simulink model "fft32kpt_ssr32_float"  (R2024a)
settings: Solver=VariableStepAuto  StartTime=0.0  StopTime=sample_period*N*6  RelTol=1e-3
PreLoadFcn:
  | clk_freq = 570e6;
  | SSR=32; % transpose block SSR settings...
  | sample_period = 1/(SSR*clk_freq);
  | N=32768; % fft point size
  | binw=(1/sample_period) / (2*N); % bin width
  | bin_freq = 2*pi*3*binw+pi*binw; % sin, cos freq centered in channel
  | 
  | % for transpose block
  | DATA_WIDTH=32;
  | M=32;
  | N1=N/M;
  | MEM_STYLE=4; % MEM OPTIONS: 4 - ULTRA, 0 - AUTO, 1 - BRAM, 5 - MIXED
InitFcn:
  | clk_freq = 570e6;
  | SSR=32; % transpose block SSR settings...
  | sample_period = 1/(SSR*clk_freq);
  | N=32768; % fft point size
  | binw=(1/sample_period) / (2*N); % bin width
  | bin_freq = 2*pi*3*binw+pi*binw; % sin, cos freq centered in channel
  | 
  | % for transpose block
  | DATA_WIDTH=32;
  | M=32;
  | N1=N/M;
  | MEM_STYLE=4; % MEM OPTIONS: 4 - ULTRA, 0 - AUTO, 1 - BRAM, 5 - MIXED
undefined symbols (not defined in the file or in its folder): None, S, vsva2197, xcvc1902
libraries: hdlBasic x139, aieBasic x95, aieUtilities x32, aieDSP x32, hdlUtilities x32, matrix_library x32, hdlSSR x12, hdlDSPIP x1, simulink x1, dspxfrm3 x1, vmcUtilities x1
(part 2 of 4)

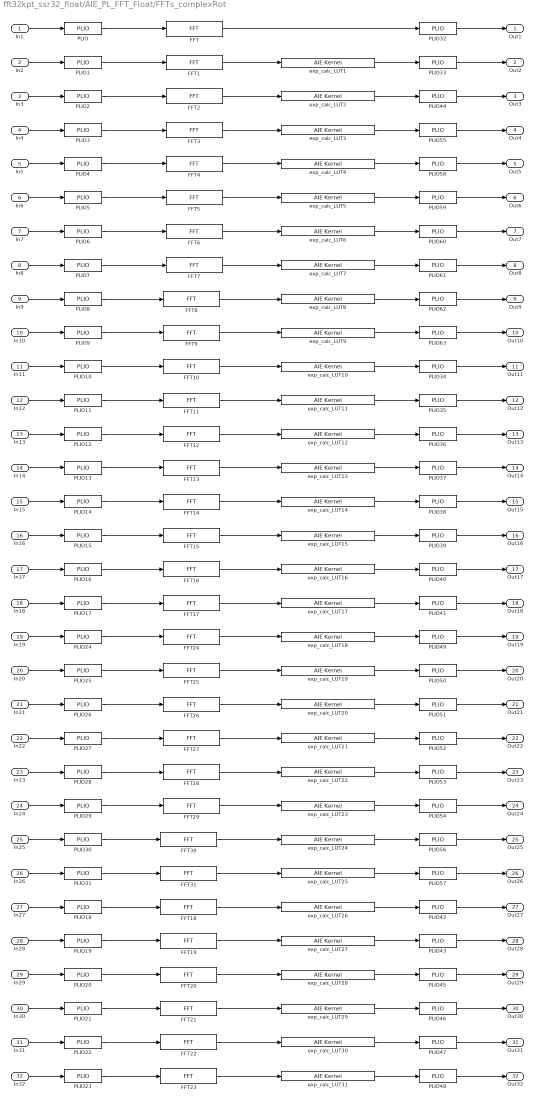
== system fft32kpt_ssr32_float/AIE_PL_FFT_Float/FFTs_complexRot ==
  In1 : Inport
  In2 : Inport  Port=2
  In3 : Inport  Port=3
  In4 : Inport  Port=4
  In5 : Inport  Port=5
  In6 : Inport  Port=6
  In7 : Inport  Port=7
  In8 : Inport  Port=8
  In9 : Inport  Port=9
  In10 : Inport  Port=10
  In11 : Inport  Port=11
  In12 : Inport  Port=12
  In13 : Inport  Port=13
  In14 : Inport  Port=14
  In15 : Inport  Port=15
  In16 : Inport  Port=16
  In17 : Inport  Port=17
  In18 : Inport  Port=18
  In19 : Inport  Port=19
  In20 : Inport  Port=20
  In21 : Inport  Port=21
  In22 : Inport  Port=22
  In23 : Inport  Port=23
  In24 : Inport  Port=24
  In25 : Inport  Port=25
  In26 : Inport  Port=26
  In27 : Inport  Port=27
  In28 : Inport  Port=28
  In29 : Inport  Port=29
  In30 : Inport  Port=30
  In31 : Inport  Port=31
  In32 : Inport  Port=32
  FFT{,1..31} (32 alike) : aieDSP/FFT  AIE_VARIANT=1  data_type=cfloat  data_out_type=cfloat  twiddle_type=cfloat  point_size=N/32  input_window_size=N/32  shift_val=0  rnd_mode=Round symmetrical to infinity  sat_mode=0-None  ssr=1  twiddle_mode=0  use_ssr_widget_kernels=off  casc_length=3  transform_fft_nifft=1  TP_API=0  TP_DYN_PT_SIZE=0  blockJsonConstraints=[]  blockJsonConstraintsInternal=[]  spec=vmc_fft.json  SerializedMaskParamNames=[]  SerializedMaskParamValues=[]  SerializedMaskParamVisibilities=[]  block_type=FFT  SerializedMaskParamDataypes=uint|typename|typename|typename|uint|uint|uint|uint|uint|uint|uint|uint|uint|uint|uint|uint  SerializedMaskParamEnumStrArr=0|0|0|0|0|0|0|Round to positive infinity,Round to negative infinity,Round symmetrical to infinity,Round symmetrical to zero,Round convergent to even,Round convergent to odd|0-None,1-Asymmetric,3-Symmetric|0|0|0|0|0|0|0  SerializedMaskParamEnumValArr=0|0|0|0|0|0|0|2,3,4,5,6,7|0,1,3|0|0|0|0|0|0|0  SerializedMaskParamVectorArr=0|0|0|0|0|0|0|0|0|0|0|0|0|0|0|0  SerializedMaskParamKeys=AIE_VARIANT|TT_DATA|TT_OUT_DATA|TT_TWIDDLE|TP_POINT_SIZE|TP_WINDOW_VSIZE|TP_SHIFT|TP_RND|TP_SAT|TP_PARALLEL_POWER|TP_TWIDDLE_MODE|TP_USE_WIDGETS|TP_CASC_LEN|TP_FFT_NIFFT|TP_API|TP_DYN_PT_SIZE
  PLIO{,1..63} (64 alike) : aieBasic/PLIO  PlioWidth=64  PlioFreqSpec=on  PlioFreq=clk_freq/1e6  ColLocation=0  channel=0  blockJsonConstraints=[]  deprecateConstraints=0
  exp_calc_LUT1 : aieBasic/AIE Kernel  KernelAllAttrs=|  PortNames={'cb_input1'; 'cb_output1'}  PortSerializedTypes={'{Q2{R{Tadf::input_buffer{1{t{Scfloat}}}}}}'; '{Q2{P{Toutput_stream{1{t{Scfloat}}}}}}'}  PortWindowSizes={1.024000000000000000e+03, 0.000000000000000000e+00}  PortWindowMargins={0.000000000000000000e+00, 0.000000000000000000e+00}  PortSynchronicities={'sync', 'auto'}  PortSignalSizes={0.000000000000000000e+00; 1.024000000000000000e+03}  FunctionTemplateSpecKind=implicit  FunctionTemplateParamNames={'PHASE_INDEX'}  FunctionTemplateParamKinds={'nontype'}  FunctionTemplateParamTypes={'unsigned int'}  FunctionTemplateParamValues={'1'}  FunctionIndex=1  FunctionTabVisible=on  FunctionTemplateParamsVisible=on  FunctionDeclTypeOptions=|  FunctionDecl=|  FunctionTemplateParams={ 'PHASE_INDEX', 'unsigned int', '1' }  FunctionTemplateParamsEnables={'off', 'off', 'on'}  PortAttrs={ 'input', 'cb_input1', 'adf::input_buffer< cfloat > & restrict', '1024', '0', 'sync', ''; 'output', 'cb_output1', 'output_stream_cfloat * restrict', '', '', '', '1024' }  PortAttrsEnables={'off', 'off', 'off', 'on', 'off', 'off', 'off';'off', 'off', 'off', 'off', 'off', 'off', 'on'}  SampleTime=-1  KernelHeaderFile=exp_calc_float.h  KernelFunction=exp_calc_float_lookup  KernelSourceFile=exp_calc_float.cc  KernelSearchPaths={}  PreProcOptions={}  blockJsonConstraints=[]
      KernelAllAttrs=|
      | s[12;12;9;9;19;14;21;23;21;23;24;21;15;17;12;24;26;26;26;27;28;9;21;23;23;23;24;25;14;19;19;29]@FunctionNameDeclFileNamePortNamesPortTypesPortSerializedTypesPortDirectionsPortWindowSizeEnablesPortWindowMarginEnablesPortBufferSizeEnablesPortBufferMarginEnablesPortSynchronicityEnablesPortSignalSizeEnablesPortBufferSizesPortBufferMarginsFunctionDeclFunctionTemplateSpecKindFunctionTemplateParamNamesFunctionTemplateParamKindsFunctionTemplateParamTypesFunctionTemplateParamValuesFunctionTemplateParamEnablesClassDeclClassTemplateSpecKindClassTemplateParamNamesClassTemplateParamKindsClassTemplateParamTypesClassTemplateParamValuesClassTemplateParamEnablesClassCtorDeclsClassCtorParamNamesClassCtorParamTypesClassCtorParamSerializedTypes[1 1]@C[32 1]@t21@exp_calc_float_lookupt22@../../exp_calc_float.hC[2 1]@t9@cb_input1t10@cb_output1C[2 1]@t38@adf::input_buffer< cfloat > & restrictt31@output_stream_cfloat * restrictC[2 1]@t42@{Q2{R{Tadf::input_buffer{1{t{Scfloat}}}}}}t38@{Q2{P{Toutput_stream{1{t{Scfloat}}}}}}C[2 1]@t5@inputt6@outputC[2 1]@l1@l0@C[2 1]@l1@l0@C[2 1]@l1@l0@C[2 1]@l0@l0@C[2 1]@l1@l0@C[2 1]@l0@l1@C[2 1]@nnC[2 1]@nnt159@template < unsigned int PHASE_INDEX > 
      | void exp_calc_float_lookup(adf::input_buffer< cfloat > & restrict cb_input1, output_stream_cfloat * restrict cb_output1)t8@implicitC[1 1]@t11@PHASE_INDEXC[1 1]@t7@nontypeC[1 1]@t12@unsigned intC[1 1]@nC[1 1]@l1@nne[0 1]@e[0 1]@e[0 1]@e[0 1]@e[0 1]@e[0 1]@e[0 1]@e[0 1]@e[0 1]@
      FunctionDeclTypeOptions=|
      | C[1 1]@t160@template < unsigned int PHASE_INDEX > 
      | void exp_calc_float_lookup(adf::input_buffer< cfloat > && restrict cb_input1, output_stream_cfloat * restrict cb_output1)
      FunctionDecl=|
      | template < unsigned int PHASE_INDEX > 
      | void exp_calc_float_lookup(adf::input_buffer< cfloat > && restrict cb_input1, output_stream_cfloat * restrict cb_output1)
  exp_calc_LUT10 : aieBasic/AIE Kernel  KernelAllAttrs=|  PortNames={'cb_input1'; 'cb_output1'}  PortSerializedTypes={'{Q2{R{Tadf::input_buffer{1{t{Scfloat}}}}}}'; '{Q2{P{Toutput_stream{1{t{Scfloat}}}}}}'}  PortWindowSizes={1.024000000000000000e+03, 0.000000000000000000e+00}  PortWindowMargins={0.000000000000000000e+00, 0.000000000000000000e+00}  PortSynchronicities={'sync', 'auto'}  PortSignalSizes={0.000000000000000000e+00; 1.024000000000000000e+03}  FunctionTemplateSpecKind=implicit  FunctionTemplateParamNames={'PHASE_INDEX'}  FunctionTemplateParamKinds={'nontype'}  FunctionTemplateParamTypes={'unsigned int'}  FunctionTemplateParamValues={'10'}  FunctionIndex=1  FunctionTabVisible=on  FunctionTemplateParamsVisible=on  FunctionDeclTypeOptions=|  FunctionDecl=|  FunctionTemplateParams={ 'PHASE_INDEX', 'unsigned int', '10' }  FunctionTemplateParamsEnables={'off', 'off', 'on'}  PortAttrs={ 'input', 'cb_input1', 'adf::input_buffer< cfloat > & restrict', '1024', '0', 'sync', ''; 'output', 'cb_output1', 'output_stream_cfloat * restrict', '', '', '', '1024' }  PortAttrsEnables={'off', 'off', 'off', 'on', 'off', 'off', 'off';'off', 'off', 'off', 'off', 'off', 'off', 'on'}  SampleTime=-1  KernelHeaderFile=exp_calc_float.h  KernelFunction=exp_calc_float_lookup  KernelSourceFile=exp_calc_float.cc  KernelSearchPaths={}  PreProcOptions={}  blockJsonConstraints=[]
      KernelAllAttrs=|
      | s[12;12;9;9;19;14;21;23;21;23;24;21;15;17;12;24;26;26;26;27;28;9;21;23;23;23;24;25;14;19;19;29]@FunctionNameDeclFileNamePortNamesPortTypesPortSerializedTypesPortDirectionsPortWindowSizeEnablesPortWindowMarginEnablesPortBufferSizeEnablesPortBufferMarginEnablesPortSynchronicityEnablesPortSignalSizeEnablesPortBufferSizesPortBufferMarginsFunctionDeclFunctionTemplateSpecKindFunctionTemplateParamNamesFunctionTemplateParamKindsFunctionTemplateParamTypesFunctionTemplateParamValuesFunctionTemplateParamEnablesClassDeclClassTemplateSpecKindClassTemplateParamNamesClassTemplateParamKindsClassTemplateParamTypesClassTemplateParamValuesClassTemplateParamEnablesClassCtorDeclsClassCtorParamNamesClassCtorParamTypesClassCtorParamSerializedTypes[1 1]@C[32 1]@t21@exp_calc_float_lookupt22@../../exp_calc_float.hC[2 1]@t9@cb_input1t10@cb_output1C[2 1]@t38@adf::input_buffer< cfloat > & restrictt31@output_stream_cfloat * restrictC[2 1]@t42@{Q2{R{Tadf::input_buffer{1{t{Scfloat}}}}}}t38@{Q2{P{Toutput_stream{1{t{Scfloat}}}}}}C[2 1]@t5@inputt6@outputC[2 1]@l1@l0@C[2 1]@l1@l0@C[2 1]@l1@l0@C[2 1]@l0@l0@C[2 1]@l1@l0@C[2 1]@l0@l1@C[2 1]@nnC[2 1]@nnt159@template < unsigned int PHASE_INDEX > 
      | void exp_calc_float_lookup(adf::input_buffer< cfloat > & restrict cb_input1, output_stream_cfloat * restrict cb_output1)t8@implicitC[1 1]@t11@PHASE_INDEXC[1 1]@t7@nontypeC[1 1]@t12@unsigned intC[1 1]@nC[1 1]@l1@nne[0 1]@e[0 1]@e[0 1]@e[0 1]@e[0 1]@e[0 1]@e[0 1]@e[0 1]@e[0 1]@
      FunctionDeclTypeOptions=|
      | C[1 1]@t160@template < unsigned int PHASE_INDEX > 
      | void exp_calc_float_lookup(adf::input_buffer< cfloat > && restrict cb_input1, output_stream_cfloat * restrict cb_output1)
      FunctionDecl=|
      | template < unsigned int PHASE_INDEX > 
      | void exp_calc_float_lookup(adf::input_buffer< cfloat > && restrict cb_input1, output_stream_cfloat * restrict cb_output1)
  exp_calc_LUT11 : aieBasic/AIE Kernel  KernelAllAttrs=|  PortNames={'cb_input1'; 'cb_output1'}  PortSerializedTypes={'{Q2{R{Tadf::input_buffer{1{t{Scfloat}}}}}}'; '{Q2{P{Toutput_stream{1{t{Scfloat}}}}}}'}  PortWindowSizes={1.024000000000000000e+03, 0.000000000000000000e+00}  PortWindowMargins={0.000000000000000000e+00, 0.000000000000000000e+00}  PortSynchronicities={'sync', 'auto'}  PortSignalSizes={0.000000000000000000e+00; 1.024000000000000000e+03}  FunctionTemplateSpecKind=implicit  FunctionTemplateParamNames={'PHASE_INDEX'}  FunctionTemplateParamKinds={'nontype'}  FunctionTemplateParamTypes={'unsigned int'}  FunctionTemplateParamValues={'11'}  FunctionIndex=1  FunctionTabVisible=on  FunctionTemplateParamsVisible=on  FunctionDeclTypeOptions=|  FunctionDecl=|  FunctionTemplateParams={ 'PHASE_INDEX', 'unsigned int', '11' }  FunctionTemplateParamsEnables={'off', 'off', 'on'}  PortAttrs={ 'input', 'cb_input1', 'adf::input_buffer< cfloat > & restrict', '1024', '0', 'sync', ''; 'output', 'cb_output1', 'output_stream_cfloat * restrict', '', '', '', '1024' }  PortAttrsEnables={'off', 'off', 'off', 'on', 'off', 'off', 'off';'off', 'off', 'off', 'off', 'off', 'off', 'on'}  SampleTime=-1  KernelHeaderFile=exp_calc_float.h  KernelFunction=exp_calc_float_lookup  KernelSourceFile=exp_calc_float.cc  KernelSearchPaths={}  PreProcOptions={}  blockJsonConstraints=[]
      KernelAllAttrs=|
      | s[12;12;9;9;19;14;21;23;21;23;24;21;15;17;12;24;26;26;26;27;28;9;21;23;23;23;24;25;14;19;19;29]@FunctionNameDeclFileNamePortNamesPortTypesPortSerializedTypesPortDirectionsPortWindowSizeEnablesPortWindowMarginEnablesPortBufferSizeEnablesPortBufferMarginEnablesPortSynchronicityEnablesPortSignalSizeEnablesPortBufferSizesPortBufferMarginsFunctionDeclFunctionTemplateSpecKindFunctionTemplateParamNamesFunctionTemplateParamKindsFunctionTemplateParamTypesFunctionTemplateParamValuesFunctionTemplateParamEnablesClassDeclClassTemplateSpecKindClassTemplateParamNamesClassTemplateParamKindsClassTemplateParamTypesClassTemplateParamValuesClassTemplateParamEnablesClassCtorDeclsClassCtorParamNamesClassCtorParamTypesClassCtorParamSerializedTypes[1 1]@C[32 1]@t21@exp_calc_float_lookupt22@../../exp_calc_float.hC[2 1]@t9@cb_input1t10@cb_output1C[2 1]@t38@adf::input_buffer< cfloat > & restrictt31@output_stream_cfloat * restrictC[2 1]@t42@{Q2{R{Tadf::input_buffer{1{t{Scfloat}}}}}}t38@{Q2{P{Toutput_stream{1{t{Scfloat}}}}}}C[2 1]@t5@inputt6@outputC[2 1]@l1@l0@C[2 1]@l1@l0@C[2 1]@l1@l0@C[2 1]@l0@l0@C[2 1]@l1@l0@C[2 1]@l0@l1@C[2 1]@nnC[2 1]@nnt159@template < unsigned int PHASE_INDEX > 
      | void exp_calc_float_lookup(adf::input_buffer< cfloat > & restrict cb_input1, output_stream_cfloat * restrict cb_output1)t8@implicitC[1 1]@t11@PHASE_INDEXC[1 1]@t7@nontypeC[1 1]@t12@unsigned intC[1 1]@nC[1 1]@l1@nne[0 1]@e[0 1]@e[0 1]@e[0 1]@e[0 1]@e[0 1]@e[0 1]@e[0 1]@e[0 1]@
      FunctionDeclTypeOptions=|
      | C[1 1]@t160@template < unsigned int PHASE_INDEX > 
      | void exp_calc_float_lookup(adf::input_buffer< cfloat > && restrict cb_input1, output_stream_cfloat * restrict cb_output1)
      FunctionDecl=|
      | template < unsigned int PHASE_INDEX > 
      | void exp_calc_float_lookup(adf::input_buffer< cfloat > && restrict cb_input1, output_stream_cfloat * restrict cb_output1)
  exp_calc_LUT12 : aieBasic/AIE Kernel  KernelAllAttrs=|  PortNames={'cb_input1'; 'cb_output1'}  PortSerializedTypes={'{Q2{R{Tadf::input_buffer{1{t{Scfloat}}}}}}'; '{Q2{P{Toutput_stream{1{t{Scfloat}}}}}}'}  PortWindowSizes={1.024000000000000000e+03, 0.000000000000000000e+00}  PortWindowMargins={0.000000000000000000e+00, 0.000000000000000000e+00}  PortSynchronicities={'sync', 'auto'}  PortSignalSizes={0.000000000000000000e+00; 1.024000000000000000e+03}  FunctionTemplateSpecKind=implicit  FunctionTemplateParamNames={'PHASE_INDEX'}  FunctionTemplateParamKinds={'nontype'}  FunctionTemplateParamTypes={'unsigned int'}  FunctionTemplateParamValues={'12'}  FunctionIndex=1  FunctionTabVisible=on  FunctionTemplateParamsVisible=on  FunctionDeclTypeOptions=|  FunctionDecl=|  FunctionTemplateParams={ 'PHASE_INDEX', 'unsigned int', '12' }  FunctionTemplateParamsEnables={'off', 'off', 'on'}  PortAttrs={ 'input', 'cb_input1', 'adf::input_buffer< cfloat > & restrict', '1024', '0', 'sync', ''; 'output', 'cb_output1', 'output_stream_cfloat * restrict', '', '', '', '1024' }  PortAttrsEnables={'off', 'off', 'off', 'on', 'off', 'off', 'off';'off', 'off', 'off', 'off', 'off', 'off', 'on'}  SampleTime=-1  KernelHeaderFile=exp_calc_float.h  KernelFunction=exp_calc_float_lookup  KernelSourceFile=exp_calc_float.cc  KernelSearchPaths={}  PreProcOptions={}  blockJsonConstraints=[]
      KernelAllAttrs=|
      | s[12;12;9;9;19;14;21;23;21;23;24;21;15;17;12;24;26;26;26;27;28;9;21;23;23;23;24;25;14;19;19;29]@FunctionNameDeclFileNamePortNamesPortTypesPortSerializedTypesPortDirectionsPortWindowSizeEnablesPortWindowMarginEnablesPortBufferSizeEnablesPortBufferMarginEnablesPortSynchronicityEnablesPortSignalSizeEnablesPortBufferSizesPortBufferMarginsFunctionDeclFunctionTemplateSpecKindFunctionTemplateParamNamesFunctionTemplateParamKindsFunctionTemplateParamTypesFunctionTemplateParamValuesFunctionTemplateParamEnablesClassDeclClassTemplateSpecKindClassTemplateParamNamesClassTemplateParamKindsClassTemplateParamTypesClassTemplateParamValuesClassTemplateParamEnablesClassCtorDeclsClassCtorParamNamesClassCtorParamTypesClassCtorParamSerializedTypes[1 1]@C[32 1]@t21@exp_calc_float_lookupt22@../../exp_calc_float.hC[2 1]@t9@cb_input1t10@cb_output1C[2 1]@t38@adf::input_buffer< cfloat > & restrictt31@output_stream_cfloat * restrictC[2 1]@t42@{Q2{R{Tadf::input_buffer{1{t{Scfloat}}}}}}t38@{Q2{P{Toutput_stream{1{t{Scfloat}}}}}}C[2 1]@t5@inputt6@outputC[2 1]@l1@l0@C[2 1]@l1@l0@C[2 1]@l1@l0@C[2 1]@l0@l0@C[2 1]@l1@l0@C[2 1]@l0@l1@C[2 1]@nnC[2 1]@nnt159@template < unsigned int PHASE_INDEX > 
      | void exp_calc_float_lookup(adf::input_buffer< cfloat > & restrict cb_input1, output_stream_cfloat * restrict cb_output1)t8@implicitC[1 1]@t11@PHASE_INDEXC[1 1]@t7@nontypeC[1 1]@t12@unsigned intC[1 1]@nC[1 1]@l1@nne[0 1]@e[0 1]@e[0 1]@e[0 1]@e[0 1]@e[0 1]@e[0 1]@e[0 1]@e[0 1]@
      FunctionDeclTypeOptions=|
      | C[1 1]@t160@template < unsigned int PHASE_INDEX > 
      | void exp_calc_float_lookup(adf::input_buffer< cfloat > && restrict cb_input1, output_stream_cfloat * restrict cb_output1)
      FunctionDecl=|
      | template < unsigned int PHASE_INDEX > 
      | void exp_calc_float_lookup(adf::input_buffer< cfloat > && restrict cb_input1, output_stream_cfloat * restrict cb_output1)
  exp_calc_LUT13 : aieBasic/AIE Kernel  KernelAllAttrs=|  PortNames={'cb_input1'; 'cb_output1'}  PortSerializedTypes={'{Q2{R{Tadf::input_buffer{1{t{Scfloat}}}}}}'; '{Q2{P{Toutput_stream{1{t{Scfloat}}}}}}'}  PortWindowSizes={1.024000000000000000e+03, 0.000000000000000000e+00}  PortWindowMargins={0.000000000000000000e+00, 0.000000000000000000e+00}  PortSynchronicities={'sync', 'auto'}  PortSignalSizes={0.000000000000000000e+00; 1.024000000000000000e+03}  FunctionTemplateSpecKind=implicit  FunctionTemplateParamNames={'PHASE_INDEX'}  FunctionTemplateParamKinds={'nontype'}  FunctionTemplateParamTypes={'unsigned int'}  FunctionTemplateParamValues={'13'}  FunctionIndex=1  FunctionTabVisible=on  FunctionTemplateParamsVisible=on  FunctionDeclTypeOptions=|  FunctionDecl=|  FunctionTemplateParams={ 'PHASE_INDEX', 'unsigned int', '13' }  FunctionTemplateParamsEnables={'off', 'off', 'on'}  PortAttrs={ 'input', 'cb_input1', 'adf::input_buffer< cfloat > & restrict', '1024', '0', 'sync', ''; 'output', 'cb_output1', 'output_stream_cfloat * restrict', '', '', '', '1024' }  PortAttrsEnables={'off', 'off', 'off', 'on', 'off', 'off', 'off';'off', 'off', 'off', 'off', 'off', 'off', 'on'}  SampleTime=-1  KernelHeaderFile=exp_calc_float.h  KernelFunction=exp_calc_float_lookup  KernelSourceFile=exp_calc_float.cc  KernelSearchPaths={}  PreProcOptions={}  blockJsonConstraints=[]
      KernelAllAttrs=|
      | s[12;12;9;9;19;14;21;23;21;23;24;21;15;17;12;24;26;26;26;27;28;9;21;23;23;23;24;25;14;19;19;29]@FunctionNameDeclFileNamePortNamesPortTypesPortSerializedTypesPortDirectionsPortWindowSizeEnablesPortWindowMarginEnablesPortBufferSizeEnablesPortBufferMarginEnablesPortSynchronicityEnablesPortSignalSizeEnablesPortBufferSizesPortBufferMarginsFunctionDeclFunctionTemplateSpecKindFunctionTemplateParamNamesFunctionTemplateParamKindsFunctionTemplateParamTypesFunctionTemplateParamValuesFunctionTemplateParamEnablesClassDeclClassTemplateSpecKindClassTemplateParamNamesClassTemplateParamKindsClassTemplateParamTypesClassTemplateParamValuesClassTemplateParamEnablesClassCtorDeclsClassCtorParamNamesClassCtorParamTypesClassCtorParamSerializedTypes[1 1]@C[32 1]@t21@exp_calc_float_lookupt22@../../exp_calc_float.hC[2 1]@t9@cb_input1t10@cb_output1C[2 1]@t38@adf::input_buffer< cfloat > & restrictt31@output_stream_cfloat * restrictC[2 1]@t42@{Q2{R{Tadf::input_buffer{1{t{Scfloat}}}}}}t38@{Q2{P{Toutput_stream{1{t{Scfloat}}}}}}C[2 1]@t5@inputt6@outputC[2 1]@l1@l0@C[2 1]@l1@l0@C[2 1]@l1@l0@C[2 1]@l0@l0@C[2 1]@l1@l0@C[2 1]@l0@l1@C[2 1]@nnC[2 1]@nnt159@template < unsigned int PHASE_INDEX > 
      | void exp_calc_float_lookup(adf::input_buffer< cfloat > & restrict cb_input1, output_stream_cfloat * restrict cb_output1)t8@implicitC[1 1]@t11@PHASE_INDEXC[1 1]@t7@nontypeC[1 1]@t12@unsigned intC[1 1]@nC[1 1]@l1@nne[0 1]@e[0 1]@e[0 1]@e[0 1]@e[0 1]@e[0 1]@e[0 1]@e[0 1]@e[0 1]@
      FunctionDeclTypeOptions=|
      | C[1 1]@t160@template < unsigned int PHASE_INDEX > 
      | void exp_calc_float_lookup(adf::input_buffer< cfloat > && restrict cb_input1, output_stream_cfloat * restrict cb_output1)
      FunctionDecl=|
      | template < unsigned int PHASE_INDEX > 
      | void exp_calc_float_lookup(adf::input_buffer< cfloat > && restrict cb_input1, output_stream_cfloat * restrict cb_output1)
  exp_calc_LUT14 : aieBasic/AIE Kernel  KernelAllAttrs=|  PortNames={'cb_input1'; 'cb_output1'}  PortSerializedTypes={'{Q2{R{Tadf::input_buffer{1{t{Scfloat}}}}}}'; '{Q2{P{Toutput_stream{1{t{Scfloat}}}}}}'}  PortWindowSizes={1.024000000000000000e+03, 0.000000000000000000e+00}  PortWindowMargins={0.000000000000000000e+00, 0.000000000000000000e+00}  PortSynchronicities={'sync', 'auto'}  PortSignalSizes={0.000000000000000000e+00; 1.024000000000000000e+03}  FunctionTemplateSpecKind=implicit  FunctionTemplateParamNames={'PHASE_INDEX'}  FunctionTemplateParamKinds={'nontype'}  FunctionTemplateParamTypes={'unsigned int'}  FunctionTemplateParamValues={'14'}  FunctionIndex=1  FunctionTabVisible=on  FunctionTemplateParamsVisible=on  FunctionDeclTypeOptions=|  FunctionDecl=|  FunctionTemplateParams={ 'PHASE_INDEX', 'unsigned int', '14' }  FunctionTemplateParamsEnables={'off', 'off', 'on'}  PortAttrs={ 'input', 'cb_input1', 'adf::input_buffer< cfloat > & restrict', '1024', '0', 'sync', ''; 'output', 'cb_output1', 'output_stream_cfloat * restrict', '', '', '', '1024' }  PortAttrsEnables={'off', 'off', 'off', 'on', 'off', 'off', 'off';'off', 'off', 'off', 'off', 'off', 'off', 'on'}  SampleTime=-1  KernelHeaderFile=exp_calc_float.h  KernelFunction=exp_calc_float_lookup  KernelSourceFile=exp_calc_float.cc  KernelSearchPaths={}  PreProcOptions={}  blockJsonConstraints=[]
      KernelAllAttrs=|
      | s[12;12;9;9;19;14;21;23;21;23;24;21;15;17;12;24;26;26;26;27;28;9;21;23;23;23;24;25;14;19;19;29]@FunctionNameDeclFileNamePortNamesPortTypesPortSerializedTypesPortDirectionsPortWindowSizeEnablesPortWindowMarginEnablesPortBufferSizeEnablesPortBufferMarginEnablesPortSynchronicityEnablesPortSignalSizeEnablesPortBufferSizesPortBufferMarginsFunctionDeclFunctionTemplateSpecKindFunctionTemplateParamNamesFunctionTemplateParamKindsFunctionTemplateParamTypesFunctionTemplateParamValuesFunctionTemplateParamEnablesClassDeclClassTemplateSpecKindClassTemplateParamNamesClassTemplateParamKindsClassTemplateParamTypesClassTemplateParamValuesClassTemplateParamEnablesClassCtorDeclsClassCtorParamNamesClassCtorParamTypesClassCtorParamSerializedTypes[1 1]@C[32 1]@t21@exp_calc_float_lookupt22@../../exp_calc_float.hC[2 1]@t9@cb_input1t10@cb_output1C[2 1]@t38@adf::input_buffer< cfloat > & restrictt31@output_stream_cfloat * restrictC[2 1]@t42@{Q2{R{Tadf::input_buffer{1{t{Scfloat}}}}}}t38@{Q2{P{Toutput_stream{1{t{Scfloat}}}}}}C[2 1]@t5@inputt6@outputC[2 1]@l1@l0@C[2 1]@l1@l0@C[2 1]@l1@l0@C[2 1]@l0@l0@C[2 1]@l1@l0@C[2 1]@l0@l1@C[2 1]@nnC[2 1]@nnt159@template < unsigned int PHASE_INDEX > 
      | void exp_calc_float_lookup(adf::input_buffer< cfloat > & restrict cb_input1, output_stream_cfloat * restrict cb_output1)t8@implicitC[1 1]@t11@PHASE_INDEXC[1 1]@t7@nontypeC[1 1]@t12@unsigned intC[1 1]@nC[1 1]@l1@nne[0 1]@e[0 1]@e[0 1]@e[0 1]@e[0 1]@e[0 1]@e[0 1]@e[0 1]@e[0 1]@
      FunctionDeclTypeOptions=|
      | C[1 1]@t160@template < unsigned int PHASE_INDEX > 
      | void exp_calc_float_lookup(adf::input_buffer< cfloat > && restrict cb_input1, output_stream_cfloat * restrict cb_output1)
      FunctionDecl=|
      | template < unsigned int PHASE_INDEX > 
      | void exp_calc_float_lookup(adf::input_buffer< cfloat > && restrict cb_input1, output_stream_cfloat * restrict cb_output1)
  exp_calc_LUT15 : aieBasic/AIE Kernel  KernelAllAttrs=|  PortNames={'cb_input1'; 'cb_output1'}  PortSerializedTypes={'{Q2{R{Tadf::input_buffer{1{t{Scfloat}}}}}}'; '{Q2{P{Toutput_stream{1{t{Scfloat}}}}}}'}  PortWindowSizes={1.024000000000000000e+03, 0.000000000000000000e+00}  PortWindowMargins={0.000000000000000000e+00, 0.000000000000000000e+00}  PortSynchronicities={'sync', 'auto'}  PortSignalSizes={0.000000000000000000e+00; 1.024000000000000000e+03}  FunctionTemplateSpecKind=implicit  FunctionTemplateParamNames={'PHASE_INDEX'}  FunctionTemplateParamKinds={'nontype'}  FunctionTemplateParamTypes={'unsigned int'}  FunctionTemplateParamValues={'15'}  FunctionIndex=1  FunctionTabVisible=on  FunctionTemplateParamsVisible=on  FunctionDeclTypeOptions=|  FunctionDecl=|  FunctionTemplateParams={ 'PHASE_INDEX', 'unsigned int', '15' }  FunctionTemplateParamsEnables={'off', 'off', 'on'}  PortAttrs={ 'input', 'cb_input1', 'adf::input_buffer< cfloat > & restrict', '1024', '0', 'sync', ''; 'output', 'cb_output1', 'output_stream_cfloat * restrict', '', '', '', '1024' }  PortAttrsEnables={'off', 'off', 'off', 'on', 'off', 'off', 'off';'off', 'off', 'off', 'off', 'off', 'off', 'on'}  SampleTime=-1  KernelHeaderFile=exp_calc_float.h  KernelFunction=exp_calc_float_lookup  KernelSourceFile=exp_calc_float.cc  KernelSearchPaths={}  PreProcOptions={}  blockJsonConstraints=[]
      KernelAllAttrs=|
      | s[12;12;9;9;19;14;21;23;21;23;24;21;15;17;12;24;26;26;26;27;28;9;21;23;23;23;24;25;14;19;19;29]@FunctionNameDeclFileNamePortNamesPortTypesPortSerializedTypesPortDirectionsPortWindowSizeEnablesPortWindowMarginEnablesPortBufferSizeEnablesPortBufferMarginEnablesPortSynchronicityEnablesPortSignalSizeEnablesPortBufferSizesPortBufferMarginsFunctionDeclFunctionTemplateSpecKindFunctionTemplateParamNamesFunctionTemplateParamKindsFunctionTemplateParamTypesFunctionTemplateParamValuesFunctionTemplateParamEnablesClassDeclClassTemplateSpecKindClassTemplateParamNamesClassTemplateParamKindsClassTemplateParamTypesClassTemplateParamValuesClassTemplateParamEnablesClassCtorDeclsClassCtorParamNamesClassCtorParamTypesClassCtorParamSerializedTypes[1 1]@C[32 1]@t21@exp_calc_float_lookupt22@../../exp_calc_float.hC[2 1]@t9@cb_input1t10@cb_output1C[2 1]@t38@adf::input_buffer< cfloat > & restrictt31@output_stream_cfloat * restrictC[2 1]@t42@{Q2{R{Tadf::input_buffer{1{t{Scfloat}}}}}}t38@{Q2{P{Toutput_stream{1{t{Scfloat}}}}}}C[2 1]@t5@inputt6@outputC[2 1]@l1@l0@C[2 1]@l1@l0@C[2 1]@l1@l0@C[2 1]@l0@l0@C[2 1]@l1@l0@C[2 1]@l0@l1@C[2 1]@nnC[2 1]@nnt159@template < unsigned int PHASE_INDEX > 
      | void exp_calc_float_lookup(adf::input_buffer< cfloat > & restrict cb_input1, output_stream_cfloat * restrict cb_output1)t8@implicitC[1 1]@t11@PHASE_INDEXC[1 1]@t7@nontypeC[1 1]@t12@unsigned intC[1 1]@nC[1 1]@l1@nne[0 1]@e[0 1]@e[0 1]@e[0 1]@e[0 1]@e[0 1]@e[0 1]@e[0 1]@e[0 1]@
      FunctionDeclTypeOptions=|
      | C[1 1]@t160@template < unsigned int PHASE_INDEX > 
      | void exp_calc_float_lookup(adf::input_buffer< cfloat > && restrict cb_input1, output_stream_cfloat * restrict cb_output1)
      FunctionDecl=|
      | template < unsigned int PHASE_INDEX > 
      | void exp_calc_float_lookup(adf::input_buffer< cfloat > && restrict cb_input1, output_stream_cfloat * restrict cb_output1)
  exp_calc_LUT16 : aieBasic/AIE Kernel  KernelAllAttrs=|  PortNames={'cb_input1'; 'cb_output1'}  PortSerializedTypes={'{Q2{R{Tadf::input_buffer{1{t{Scfloat}}}}}}'; '{Q2{P{Toutput_stream{1{t{Scfloat}}}}}}'}  PortWindowSizes={1.024000000000000000e+03, 0.000000000000000000e+00}  PortWindowMargins={0.000000000000000000e+00, 0.000000000000000000e+00}  PortSynchronicities={'sync', 'auto'}  PortSignalSizes={0.000000000000000000e+00; 1.024000000000000000e+03}  FunctionTemplateSpecKind=implicit  FunctionTemplateParamNames={'PHASE_INDEX'}  FunctionTemplateParamKinds={'nontype'}  FunctionTemplateParamTypes={'unsigned int'}  FunctionTemplateParamValues={'16'}  FunctionIndex=1  FunctionTabVisible=on  FunctionTemplateParamsVisible=on  FunctionDeclTypeOptions=|  FunctionDecl=|  FunctionTemplateParams={ 'PHASE_INDEX', 'unsigned int', '16' }  FunctionTemplateParamsEnables={'off', 'off', 'on'}  PortAttrs={ 'input', 'cb_input1', 'adf::input_buffer< cfloat > & restrict', '1024', '0', 'sync', ''; 'output', 'cb_output1', 'output_stream_cfloat * restrict', '', '', '', '1024' }  PortAttrsEnables={'off', 'off', 'off', 'on', 'off', 'off', 'off';'off', 'off', 'off', 'off', 'off', 'off', 'on'}  SampleTime=-1  KernelHeaderFile=exp_calc_float.h  KernelFunction=exp_calc_float_lookup  KernelSourceFile=exp_calc_float.cc  KernelSearchPaths={}  PreProcOptions={}  blockJsonConstraints=[]
      KernelAllAttrs=|
      | s[12;12;9;9;19;14;21;23;21;23;24;21;15;17;12;24;26;26;26;27;28;9;21;23;23;23;24;25;14;19;19;29]@FunctionNameDeclFileNamePortNamesPortTypesPortSerializedTypesPortDirectionsPortWindowSizeEnablesPortWindowMarginEnablesPortBufferSizeEnablesPortBufferMarginEnablesPortSynchronicityEnablesPortSignalSizeEnablesPortBufferSizesPortBufferMarginsFunctionDeclFunctionTemplateSpecKindFunctionTemplateParamNamesFunctionTemplateParamKindsFunctionTemplateParamTypesFunctionTemplateParamValuesFunctionTemplateParamEnablesClassDeclClassTemplateSpecKindClassTemplateParamNamesClassTemplateParamKindsClassTemplateParamTypesClassTemplateParamValuesClassTemplateParamEnablesClassCtorDeclsClassCtorParamNamesClassCtorParamTypesClassCtorParamSerializedTypes[1 1]@C[32 1]@t21@exp_calc_float_lookupt22@../../exp_calc_float.hC[2 1]@t9@cb_input1t10@cb_output1C[2 1]@t38@adf::input_buffer< cfloat > & restrictt31@output_stream_cfloat * restrictC[2 1]@t42@{Q2{R{Tadf::input_buffer{1{t{Scfloat}}}}}}t38@{Q2{P{Toutput_stream{1{t{Scfloat}}}}}}C[2 1]@t5@inputt6@outputC[2 1]@l1@l0@C[2 1]@l1@l0@C[2 1]@l1@l0@C[2 1]@l0@l0@C[2 1]@l1@l0@C[2 1]@l0@l1@C[2 1]@nnC[2 1]@nnt159@template < unsigned int PHASE_INDEX > 
      | void exp_calc_float_lookup(adf::input_buffer< cfloat > & restrict cb_input1, output_stream_cfloat * restrict cb_output1)t8@implicitC[1 1]@t11@PHASE_INDEXC[1 1]@t7@nontypeC[1 1]@t12@unsigned intC[1 1]@nC[1 1]@l1@nne[0 1]@e[0 1]@e[0 1]@e[0 1]@e[0 1]@e[0 1]@e[0 1]@e[0 1]@e[0 1]@
      FunctionDeclTypeOptions=|
      | C[1 1]@t160@template < unsigned int PHASE_INDEX > 
      | void exp_calc_float_lookup(adf::input_buffer< cfloat > && restrict cb_input1, output_stream_cfloat * restrict cb_output1)
      FunctionDecl=|
      | template < unsigned int PHASE_INDEX > 
      | void exp_calc_float_lookup(adf::input_buffer< cfloat > && restrict cb_input1, output_stream_cfloat * restrict cb_output1)
  exp_calc_LUT17 : aieBasic/AIE Kernel  KernelAllAttrs=|  PortNames={'cb_input1'; 'cb_output1'}  PortSerializedTypes={'{Q2{R{Tadf::input_buffer{1{t{Scfloat}}}}}}'; '{Q2{P{Toutput_stream{1{t{Scfloat}}}}}}'}  PortWindowSizes={1.024000000000000000e+03, 0.000000000000000000e+00}  PortWindowMargins={0.000000000000000000e+00, 0.000000000000000000e+00}  PortSynchronicities={'sync', 'auto'}  PortSignalSizes={0.000000000000000000e+00; 1.024000000000000000e+03}  FunctionTemplateSpecKind=implicit  FunctionTemplateParamNames={'PHASE_INDEX'}  FunctionTemplateParamKinds={'nontype'}  FunctionTemplateParamTypes={'unsigned int'}  FunctionTemplateParamValues={'17'}  FunctionIndex=1  FunctionTabVisible=on  FunctionTemplateParamsVisible=on  FunctionDeclTypeOptions=|  FunctionDecl=|  FunctionTemplateParams={ 'PHASE_INDEX', 'unsigned int', '17' }  FunctionTemplateParamsEnables={'off', 'off', 'on'}  PortAttrs={ 'input', 'cb_input1', 'adf::input_buffer< cfloat > & restrict', '1024', '0', 'sync', ''; 'output', 'cb_output1', 'output_stream_cfloat * restrict', '', '', '', '1024' }  PortAttrsEnables={'off', 'off', 'off', 'on', 'off', 'off', 'off';'off', 'off', 'off', 'off', 'off', 'off', 'on'}  SampleTime=-1  KernelHeaderFile=exp_calc_float.h  KernelFunction=exp_calc_float_lookup  KernelSourceFile=exp_calc_float.cc  KernelSearchPaths={}  PreProcOptions={}  blockJsonConstraints=[]
      KernelAllAttrs=|
      | s[12;12;9;9;19;14;21;23;21;23;24;21;15;17;12;24;26;26;26;27;28;9;21;23;23;23;24;25;14;19;19;29]@FunctionNameDeclFileNamePortNamesPortTypesPortSerializedTypesPortDirectionsPortWindowSizeEnablesPortWindowMarginEnablesPortBufferSizeEnablesPortBufferMarginEnablesPortSynchronicityEnablesPortSignalSizeEnablesPortBufferSizesPortBufferMarginsFunctionDeclFunctionTemplateSpecKindFunctionTemplateParamNamesFunctionTemplateParamKindsFunctionTemplateParamTypesFunctionTemplateParamValuesFunctionTemplateParamEnablesClassDeclClassTemplateSpecKindClassTemplateParamNamesClassTemplateParamKindsClassTemplateParamTypesClassTemplateParamValuesClassTemplateParamEnablesClassCtorDeclsClassCtorParamNamesClassCtorParamTypesClassCtorParamSerializedTypes[1 1]@C[32 1]@t21@exp_calc_float_lookupt22@../../exp_calc_float.hC[2 1]@t9@cb_input1t10@cb_output1C[2 1]@t38@adf::input_buffer< cfloat > & restrictt31@output_stream_cfloat * restrictC[2 1]@t42@{Q2{R{Tadf::input_buffer{1{t{Scfloat}}}}}}t38@{Q2{P{Toutput_stream{1{t{Scfloat}}}}}}C[2 1]@t5@inputt6@outputC[2 1]@l1@l0@C[2 1]@l1@l0@C[2 1]@l1@l0@C[2 1]@l0@l0@C[2 1]@l1@l0@C[2 1]@l0@l1@C[2 1]@nnC[2 1]@nnt159@template < unsigned int PHASE_INDEX > 
      | void exp_calc_float_lookup(adf::input_buffer< cfloat > & restrict cb_input1, output_stream_cfloat * restrict cb_output1)t8@implicitC[1 1]@t11@PHASE_INDEXC[1 1]@t7@nontypeC[1 1]@t12@unsigned intC[1 1]@nC[1 1]@l1@nne[0 1]@e[0 1]@e[0 1]@e[0 1]@e[0 1]@e[0 1]@e[0 1]@e[0 1]@e[0 1]@
      FunctionDeclTypeOptions=|
      | C[1 1]@t160@template < unsigned int PHASE_INDEX > 
      | void exp_calc_float_lookup(adf::input_buffer< cfloat > && restrict cb_input1, output_stream_cfloat * restrict cb_output1)
      FunctionDecl=|
      | template < unsigned int PHASE_INDEX > 
      | void exp_calc_float_lookup(adf::input_buffer< cfloat > && restrict cb_input1, output_stream_cfloat * restrict cb_output1)
  exp_calc_LUT18 : aieBasic/AIE Kernel  KernelAllAttrs=|  PortNames={'cb_input1'; 'cb_output1'}  PortSerializedTypes={'{Q2{R{Tadf::input_buffer{1{t{Scfloat}}}}}}'; '{Q2{P{Toutput_stream{1{t{Scfloat}}}}}}'}  PortWindowSizes={1.024000000000000000e+03, 0.000000000000000000e+00}  PortWindowMargins={0.000000000000000000e+00, 0.000000000000000000e+00}  PortSynchronicities={'sync', 'auto'}  PortSignalSizes={0.000000000000000000e+00; 1.024000000000000000e+03}  FunctionTemplateSpecKind=implicit  FunctionTemplateParamNames={'PHASE_INDEX'}  FunctionTemplateParamKinds={'nontype'}  FunctionTemplateParamTypes={'unsigned int'}  FunctionTemplateParamValues={'18'}  FunctionIndex=1  FunctionTabVisible=on  FunctionTemplateParamsVisible=on  FunctionDeclTypeOptions=|  FunctionDecl=|  FunctionTemplateParams={ 'PHASE_INDEX', 'unsigned int', '18' }  FunctionTemplateParamsEnables={'off', 'off', 'on'}  PortAttrs={ 'input', 'cb_input1', 'adf::input_buffer< cfloat > & restrict', '1024', '0', 'sync', ''; 'output', 'cb_output1', 'output_stream_cfloat * restrict', '', '', '', '1024' }  PortAttrsEnables={'off', 'off', 'off', 'on', 'off', 'off', 'off';'off', 'off', 'off', 'off', 'off', 'off', 'on'}  SampleTime=-1  KernelHeaderFile=exp_calc_float.h  KernelFunction=exp_calc_float_lookup  KernelSourceFile=exp_calc_float.cc  KernelSearchPaths={}  PreProcOptions={}  blockJsonConstraints=[]
      KernelAllAttrs=|
      | s[12;12;9;9;19;14;21;23;21;23;24;21;15;17;12;24;26;26;26;27;28;9;21;23;23;23;24;25;14;19;19;29]@FunctionNameDeclFileNamePortNamesPortTypesPortSerializedTypesPortDirectionsPortWindowSizeEnablesPortWindowMarginEnablesPortBufferSizeEnablesPortBufferMarginEnablesPortSynchronicityEnablesPortSignalSizeEnablesPortBufferSizesPortBufferMarginsFunctionDeclFunctionTemplateSpecKindFunctionTemplateParamNamesFunctionTemplateParamKindsFunctionTemplateParamTypesFunctionTemplateParamValuesFunctionTemplateParamEnablesClassDeclClassTemplateSpecKindClassTemplateParamNamesClassTemplateParamKindsClassTemplateParamTypesClassTemplateParamValuesClassTemplateParamEnablesClassCtorDeclsClassCtorParamNamesClassCtorParamTypesClassCtorParamSerializedTypes[1 1]@C[32 1]@t21@exp_calc_float_lookupt22@../../exp_calc_float.hC[2 1]@t9@cb_input1t10@cb_output1C[2 1]@t38@adf::input_buffer< cfloat > & restrictt31@output_stream_cfloat * restrictC[2 1]@t42@{Q2{R{Tadf::input_buffer{1{t{Scfloat}}}}}}t38@{Q2{P{Toutput_stream{1{t{Scfloat}}}}}}C[2 1]@t5@inputt6@outputC[2 1]@l1@l0@C[2 1]@l1@l0@C[2 1]@l1@l0@C[2 1]@l0@l0@C[2 1]@l1@l0@C[2 1]@l0@l1@C[2 1]@nnC[2 1]@nnt159@template < unsigned int PHASE_INDEX > 
      | void exp_calc_float_lookup(adf::input_buffer< cfloat > & restrict cb_input1, output_stream_cfloat * restrict cb_output1)t8@implicitC[1 1]@t11@PHASE_INDEXC[1 1]@t7@nontypeC[1 1]@t12@unsigned intC[1 1]@nC[1 1]@l1@nne[0 1]@e[0 1]@e[0 1]@e[0 1]@e[0 1]@e[0 1]@e[0 1]@e[0 1]@e[0 1]@
      FunctionDeclTypeOptions=|
      | C[1 1]@t160@template < unsigned int PHASE_INDEX > 
      | void exp_calc_float_lookup(adf::input_buffer< cfloat > && restrict cb_input1, output_stream_cfloat * restrict cb_output1)
      FunctionDecl=|
      | template < unsigned int PHASE_INDEX > 
      | void exp_calc_float_lookup(adf::input_buffer< cfloat > && restrict cb_input1, output_stream_cfloat * restrict cb_output1)
  exp_calc_LUT19 : aieBasic/AIE Kernel  KernelAllAttrs=|  PortNames={'cb_input1'; 'cb_output1'}  PortSerializedTypes={'{Q2{R{Tadf::input_buffer{1{t{Scfloat}}}}}}'; '{Q2{P{Toutput_stream{1{t{Scfloat}}}}}}'}  PortWindowSizes={1.024000000000000000e+03, 0.000000000000000000e+00}  PortWindowMargins={0.000000000000000000e+00, 0.000000000000000000e+00}  PortSynchronicities={'sync', 'auto'}  PortSignalSizes={0.000000000000000000e+00; 1.024000000000000000e+03}  FunctionTemplateSpecKind=implicit  FunctionTemplateParamNames={'PHASE_INDEX'}  FunctionTemplateParamKinds={'nontype'}  FunctionTemplateParamTypes={'unsigned int'}  FunctionTemplateParamValues={'19'}  FunctionIndex=1  FunctionTabVisible=on  FunctionTemplateParamsVisible=on  FunctionDeclTypeOptions=|  FunctionDecl=|  FunctionTemplateParams={ 'PHASE_INDEX', 'unsigned int', '19' }  FunctionTemplateParamsEnables={'off', 'off', 'on'}  PortAttrs={ 'input', 'cb_input1', 'adf::input_buffer< cfloat > & restrict', '1024', '0', 'sync', ''; 'output', 'cb_output1', 'output_stream_cfloat * restrict', '', '', '', '1024' }  PortAttrsEnables={'off', 'off', 'off', 'on', 'off', 'off', 'off';'off', 'off', 'off', 'off', 'off', 'off', 'on'}  SampleTime=-1  KernelHeaderFile=exp_calc_float.h  KernelFunction=exp_calc_float_lookup  KernelSourceFile=exp_calc_float.cc  KernelSearchPaths={}  PreProcOptions={}  blockJsonConstraints=[]
      KernelAllAttrs=|
      | s[12;12;9;9;19;14;21;23;21;23;24;21;15;17;12;24;26;26;26;27;28;9;21;23;23;23;24;25;14;19;19;29]@FunctionNameDeclFileNamePortNamesPortTypesPortSerializedTypesPortDirectionsPortWindowSizeEnablesPortWindowMarginEnablesPortBufferSizeEnablesPortBufferMarginEnablesPortSynchronicityEnablesPortSignalSizeEnablesPortBufferSizesPortBufferMarginsFunctionDeclFunctionTemplateSpecKindFunctionTemplateParamNamesFunctionTemplateParamKindsFunctionTemplateParamTypesFunctionTemplateParamValuesFunctionTemplateParamEnablesClassDeclClassTemplateSpecKindClassTemplateParamNamesClassTemplateParamKindsClassTemplateParamTypesClassTemplateParamValuesClassTemplateParamEnablesClassCtorDeclsClassCtorParamNamesClassCtorParamTypesClassCtorParamSerializedTypes[1 1]@C[32 1]@t21@exp_calc_float_lookupt22@../../exp_calc_float.hC[2 1]@t9@cb_input1t10@cb_output1C[2 1]@t38@adf::input_buffer< cfloat > & restrictt31@output_stream_cfloat * restrictC[2 1]@t42@{Q2{R{Tadf::input_buffer{1{t{Scfloat}}}}}}t38@{Q2{P{Toutput_stream{1{t{Scfloat}}}}}}C[2 1]@t5@inputt6@outputC[2 1]@l1@l0@C[2 1]@l1@l0@C[2 1]@l1@l0@C[2 1]@l0@l0@C[2 1]@l1@l0@C[2 1]@l0@l1@C[2 1]@nnC[2 1]@nnt159@template < unsigned int PHASE_INDEX > 
      | void exp_calc_float_lookup(adf::input_buffer< cfloat > & restrict cb_input1, output_stream_cfloat * restrict cb_output1)t8@implicitC[1 1]@t11@PHASE_INDEXC[1 1]@t7@nontypeC[1 1]@t12@unsigned intC[1 1]@nC[1 1]@l1@nne[0 1]@e[0 1]@e[0 1]@e[0 1]@e[0 1]@e[0 1]@e[0 1]@e[0 1]@e[0 1]@
      FunctionDeclTypeOptions=|
      | C[1 1]@t160@template < unsigned int PHASE_INDEX > 
      | void exp_calc_float_lookup(adf::input_buffer< cfloat > && restrict cb_input1, output_stream_cfloat * restrict cb_output1)
      FunctionDecl=|
      | template < unsigned int PHASE_INDEX > 
      | void exp_calc_float_lookup(adf::input_buffer< cfloat > && restrict cb_input1, output_stream_cfloat * restrict cb_output1)
  exp_calc_LUT2 : aieBasic/AIE Kernel  KernelAllAttrs=|  PortNames={'cb_input1'; 'cb_output1'}  PortSerializedTypes={'{Q2{R{Tadf::input_buffer{1{t{Scfloat}}}}}}'; '{Q2{P{Toutput_stream{1{t{Scfloat}}}}}}'}  PortWindowSizes={1.024000000000000000e+03, 0.000000000000000000e+00}  PortWindowMargins={0.000000000000000000e+00, 0.000000000000000000e+00}  PortSynchronicities={'sync', 'auto'}  PortSignalSizes={0.000000000000000000e+00; 1.024000000000000000e+03}  FunctionTemplateSpecKind=implicit  FunctionTemplateParamNames={'PHASE_INDEX'}  FunctionTemplateParamKinds={'nontype'}  FunctionTemplateParamTypes={'unsigned int'}  FunctionTemplateParamValues={'2'}  FunctionIndex=1  FunctionTabVisible=on  FunctionTemplateParamsVisible=on  FunctionDeclTypeOptions=|  FunctionDecl=|  FunctionTemplateParams={ 'PHASE_INDEX', 'unsigned int', '2' }  FunctionTemplateParamsEnables={'off', 'off', 'on'}  PortAttrs={ 'input', 'cb_input1', 'adf::input_buffer< cfloat > & restrict', '1024', '0', 'sync', ''; 'output', 'cb_output1', 'output_stream_cfloat * restrict', '', '', '', '1024' }  PortAttrsEnables={'off', 'off', 'off', 'on', 'off', 'off', 'off';'off', 'off', 'off', 'off', 'off', 'off', 'on'}  SampleTime=-1  KernelHeaderFile=exp_calc_float.h  KernelFunction=exp_calc_float_lookup  KernelSourceFile=exp_calc_float.cc  KernelSearchPaths={}  PreProcOptions={}  blockJsonConstraints=[]
      KernelAllAttrs=|
      | s[12;12;9;9;19;14;21;23;21;23;24;21;15;17;12;24;26;26;26;27;28;9;21;23;23;23;24;25;14;19;19;29]@FunctionNameDeclFileNamePortNamesPortTypesPortSerializedTypesPortDirectionsPortWindowSizeEnablesPortWindowMarginEnablesPortBufferSizeEnablesPortBufferMarginEnablesPortSynchronicityEnablesPortSignalSizeEnablesPortBufferSizesPortBufferMarginsFunctionDeclFunctionTemplateSpecKindFunctionTemplateParamNamesFunctionTemplateParamKindsFunctionTemplateParamTypesFunctionTemplateParamValuesFunctionTemplateParamEnablesClassDeclClassTemplateSpecKindClassTemplateParamNamesClassTemplateParamKindsClassTemplateParamTypesClassTemplateParamValuesClassTemplateParamEnablesClassCtorDeclsClassCtorParamNamesClassCtorParamTypesClassCtorParamSerializedTypes[1 1]@C[32 1]@t21@exp_calc_float_lookupt22@../../exp_calc_float.hC[2 1]@t9@cb_input1t10@cb_output1C[2 1]@t38@adf::input_buffer< cfloat > & restrictt31@output_stream_cfloat * restrictC[2 1]@t42@{Q2{R{Tadf::input_buffer{1{t{Scfloat}}}}}}t38@{Q2{P{Toutput_stream{1{t{Scfloat}}}}}}C[2 1]@t5@inputt6@outputC[2 1]@l1@l0@C[2 1]@l1@l0@C[2 1]@l1@l0@C[2 1]@l0@l0@C[2 1]@l1@l0@C[2 1]@l0@l1@C[2 1]@nnC[2 1]@nnt159@template < unsigned int PHASE_INDEX > 
      | void exp_calc_float_lookup(adf::input_buffer< cfloat > & restrict cb_input1, output_stream_cfloat * restrict cb_output1)t8@implicitC[1 1]@t11@PHASE_INDEXC[1 1]@t7@nontypeC[1 1]@t12@unsigned intC[1 1]@nC[1 1]@l1@nne[0 1]@e[0 1]@e[0 1]@e[0 1]@e[0 1]@e[0 1]@e[0 1]@e[0 1]@e[0 1]@
      FunctionDeclTypeOptions=|
      | C[1 1]@t160@template < unsigned int PHASE_INDEX > 
      | void exp_calc_float_lookup(adf::input_buffer< cfloat > && restrict cb_input1, output_stream_cfloat * restrict cb_output1)
      FunctionDecl=|
      | template < unsigned int PHASE_INDEX > 
      | void exp_calc_float_lookup(adf::input_buffer< cfloat > && restrict cb_input1, output_stream_cfloat * restrict cb_output1)
  exp_calc_LUT20 : aieBasic/AIE Kernel  KernelAllAttrs=|  PortNames={'cb_input1'; 'cb_output1'}  PortSerializedTypes={'{Q2{R{Tadf::input_buffer{1{t{Scfloat}}}}}}'; '{Q2{P{Toutput_stream{1{t{Scfloat}}}}}}'}  PortWindowSizes={1.024000000000000000e+03, 0.000000000000000000e+00}  PortWindowMargins={0.000000000000000000e+00, 0.000000000000000000e+00}  PortSynchronicities={'sync', 'auto'}  PortSignalSizes={0.000000000000000000e+00; 1.024000000000000000e+03}  FunctionTemplateSpecKind=implicit  FunctionTemplateParamNames={'PHASE_INDEX'}  FunctionTemplateParamKinds={'nontype'}  FunctionTemplateParamTypes={'unsigned int'}  FunctionTemplateParamValues={'20'}  FunctionIndex=1  FunctionTabVisible=on  FunctionTemplateParamsVisible=on  FunctionDeclTypeOptions=|  FunctionDecl=|  FunctionTemplateParams={ 'PHASE_INDEX', 'unsigned int', '20' }  FunctionTemplateParamsEnables={'off', 'off', 'on'}  PortAttrs={ 'input', 'cb_input1', 'adf::input_buffer< cfloat > & restrict', '1024', '0', 'sync', ''; 'output', 'cb_output1', 'output_stream_cfloat * restrict', '', '', '', '1024' }  PortAttrsEnables={'off', 'off', 'off', 'on', 'off', 'off', 'off';'off', 'off', 'off', 'off', 'off', 'off', 'on'}  SampleTime=-1  KernelHeaderFile=exp_calc_float.h  KernelFunction=exp_calc_float_lookup  KernelSourceFile=exp_calc_float.cc  KernelSearchPaths={}  PreProcOptions={}  blockJsonConstraints=[]
      KernelAllAttrs=|
      | s[12;12;9;9;19;14;21;23;21;23;24;21;15;17;12;24;26;26;26;27;28;9;21;23;23;23;24;25;14;19;19;29]@FunctionNameDeclFileNamePortNamesPortTypesPortSerializedTypesPortDirectionsPortWindowSizeEnablesPortWindowMarginEnablesPortBufferSizeEnablesPortBufferMarginEnablesPortSynchronicityEnablesPortSignalSizeEnablesPortBufferSizesPortBufferMarginsFunctionDeclFunctionTemplateSpecKindFunctionTemplateParamNamesFunctionTemplateParamKindsFunctionTemplateParamTypesFunctionTemplateParamValuesFunctionTemplateParamEnablesClassDeclClassTemplateSpecKindClassTemplateParamNamesClassTemplateParamKindsClassTemplateParamTypesClassTemplateParamValuesClassTemplateParamEnablesClassCtorDeclsClassCtorParamNamesClassCtorParamTypesClassCtorParamSerializedTypes[1 1]@C[32 1]@t21@exp_calc_float_lookupt22@../../exp_calc_float.hC[2 1]@t9@cb_input1t10@cb_output1C[2 1]@t38@adf::input_buffer< cfloat > & restrictt31@output_stream_cfloat * restrictC[2 1]@t42@{Q2{R{Tadf::input_buffer{1{t{Scfloat}}}}}}t38@{Q2{P{Toutput_stream{1{t{Scfloat}}}}}}C[2 1]@t5@inputt6@outputC[2 1]@l1@l0@C[2 1]@l1@l0@C[2 1]@l1@l0@C[2 1]@l0@l0@C[2 1]@l1@l0@C[2 1]@l0@l1@C[2 1]@nnC[2 1]@nnt159@template < unsigned int PHASE_INDEX > 
      | void exp_calc_float_lookup(adf::input_buffer< cfloat > & restrict cb_input1, output_stream_cfloat * restrict cb_output1)t8@implicitC[1 1]@t11@PHASE_INDEXC[1 1]@t7@nontypeC[1 1]@t12@unsigned intC[1 1]@nC[1 1]@l1@nne[0 1]@e[0 1]@e[0 1]@e[0 1]@e[0 1]@e[0 1]@e[0 1]@e[0 1]@e[0 1]@
      FunctionDeclTypeOptions=|
      | C[1 1]@t160@template < unsigned int PHASE_INDEX > 
      | void exp_calc_float_lookup(adf::input_buffer< cfloat > && restrict cb_input1, output_stream_cfloat * restrict cb_output1)
      FunctionDecl=|
      | template < unsigned int PHASE_INDEX > 
      | void exp_calc_float_lookup(adf::input_buffer< cfloat > && restrict cb_input1, output_stream_cfloat * restrict cb_output1)
  exp_calc_LUT21 : aieBasic/AIE Kernel  KernelAllAttrs=|  PortNames={'cb_input1'; 'cb_output1'}  PortSerializedTypes={'{Q2{R{Tadf::input_buffer{1{t{Scfloat}}}}}}'; '{Q2{P{Toutput_stream{1{t{Scfloat}}}}}}'}  PortWindowSizes={1.024000000000000000e+03, 0.000000000000000000e+00}  PortWindowMargins={0.000000000000000000e+00, 0.000000000000000000e+00}  PortSynchronicities={'sync', 'auto'}  PortSignalSizes={0.000000000000000000e+00; 1.024000000000000000e+03}  FunctionTemplateSpecKind=implicit  FunctionTemplateParamNames={'PHASE_INDEX'}  FunctionTemplateParamKinds={'nontype'}  FunctionTemplateParamTypes={'unsigned int'}  FunctionTemplateParamValues={'21'}  FunctionIndex=1  FunctionTabVisible=on  FunctionTemplateParamsVisible=on  FunctionDeclTypeOptions=|  FunctionDecl=|  FunctionTemplateParams={ 'PHASE_INDEX', 'unsigned int', '21' }  FunctionTemplateParamsEnables={'off', 'off', 'on'}  PortAttrs={ 'input', 'cb_input1', 'adf::input_buffer< cfloat > & restrict', '1024', '0', 'sync', ''; 'output', 'cb_output1', 'output_stream_cfloat * restrict', '', '', '', '1024' }  PortAttrsEnables={'off', 'off', 'off', 'on', 'off', 'off', 'off';'off', 'off', 'off', 'off', 'off', 'off', 'on'}  SampleTime=-1  KernelHeaderFile=exp_calc_float.h  KernelFunction=exp_calc_float_lookup  KernelSourceFile=exp_calc_float.cc  KernelSearchPaths={}  PreProcOptions={}  blockJsonConstraints=[]
      KernelAllAttrs=|
      | s[12;12;9;9;19;14;21;23;21;23;24;21;15;17;12;24;26;26;26;27;28;9;21;23;23;23;24;25;14;19;19;29]@FunctionNameDeclFileNamePortNamesPortTypesPortSerializedTypesPortDirectionsPortWindowSizeEnablesPortWindowMarginEnablesPortBufferSizeEnablesPortBufferMarginEnablesPortSynchronicityEnablesPortSignalSizeEnablesPortBufferSizesPortBufferMarginsFunctionDeclFunctionTemplateSpecKindFunctionTemplateParamNamesFunctionTemplateParamKindsFunctionTemplateParamTypesFunctionTemplateParamValuesFunctionTemplateParamEnablesClassDeclClassTemplateSpecKindClassTemplateParamNamesClassTemplateParamKindsClassTemplateParamTypesClassTemplateParamValuesClassTemplateParamEnablesClassCtorDeclsClassCtorParamNamesClassCtorParamTypesClassCtorParamSerializedTypes[1 1]@C[32 1]@t21@exp_calc_float_lookupt22@../../exp_calc_float.hC[2 1]@t9@cb_input1t10@cb_output1C[2 1]@t38@adf::input_buffer< cfloat > & restrictt31@output_stream_cfloat * restrictC[2 1]@t42@{Q2{R{Tadf::input_buffer{1{t{Scfloat}}}}}}t38@{Q2{P{Toutput_stream{1{t{Scfloat}}}}}}C[2 1]@t5@inputt6@outputC[2 1]@l1@l0@C[2 1]@l1@l0@C[2 1]@l1@l0@C[2 1]@l0@l0@C[2 1]@l1@l0@C[2 1]@l0@l1@C[2 1]@nnC[2 1]@nnt159@template < unsigned int PHASE_INDEX > 
      | void exp_calc_float_lookup(adf::input_buffer< cfloat > & restrict cb_input1, output_stream_cfloat * restrict cb_output1)t8@implicitC[1 1]@t11@PHASE_INDEXC[1 1]@t7@nontypeC[1 1]@t12@unsigned intC[1 1]@nC[1 1]@l1@nne[0 1]@e[0 1]@e[0 1]@e[0 1]@e[0 1]@e[0 1]@e[0 1]@e[0 1]@e[0 1]@
      FunctionDeclTypeOptions=|
      | C[1 1]@t160@template < unsigned int PHASE_INDEX > 
      | void exp_calc_float_lookup(adf::input_buffer< cfloat > && restrict cb_input1, output_stream_cfloat * restrict cb_output1)
      FunctionDecl=|
      | template < unsigned int PHASE_INDEX > 
      | void exp_calc_float_lookup(adf::input_buffer< cfloat > && restrict cb_input1, output_stream_cfloat * restrict cb_output1)
  exp_calc_LUT22 : aieBasic/AIE Kernel  KernelAllAttrs=|  PortNames={'cb_input1'; 'cb_output1'}  PortSerializedTypes={'{Q2{R{Tadf::input_buffer{1{t{Scfloat}}}}}}'; '{Q2{P{Toutput_stream{1{t{Scfloat}}}}}}'}  PortWindowSizes={1.024000000000000000e+03, 0.000000000000000000e+00}  PortWindowMargins={0.000000000000000000e+00, 0.000000000000000000e+00}  PortSynchronicities={'sync', 'auto'}  PortSignalSizes={0.000000000000000000e+00; 1.024000000000000000e+03}  FunctionTemplateSpecKind=implicit  FunctionTemplateParamNames={'PHASE_INDEX'}  FunctionTemplateParamKinds={'nontype'}  FunctionTemplateParamTypes={'unsigned int'}  FunctionTemplateParamValues={'22'}  FunctionIndex=1  FunctionTabVisible=on  FunctionTemplateParamsVisible=on  FunctionDeclTypeOptions=|  FunctionDecl=|  FunctionTemplateParams={ 'PHASE_INDEX', 'unsigned int', '22' }  FunctionTemplateParamsEnables={'off', 'off', 'on'}  PortAttrs={ 'input', 'cb_input1', 'adf::input_buffer< cfloat > & restrict', '1024', '0', 'sync', ''; 'output', 'cb_output1', 'output_stream_cfloat * restrict', '', '', '', '1024' }  PortAttrsEnables={'off', 'off', 'off', 'on', 'off', 'off', 'off';'off', 'off', 'off', 'off', 'off', 'off', 'on'}  SampleTime=-1  KernelHeaderFile=exp_calc_float.h  KernelFunction=exp_calc_float_lookup  KernelSourceFile=exp_calc_float.cc  KernelSearchPaths={}  PreProcOptions={}  blockJsonConstraints=[]
      KernelAllAttrs=|
      | s[12;12;9;9;19;14;21;23;21;23;24;21;15;17;12;24;26;26;26;27;28;9;21;23;23;23;24;25;14;19;19;29]@FunctionNameDeclFileNamePortNamesPortTypesPortSerializedTypesPortDirectionsPortWindowSizeEnablesPortWindowMarginEnablesPortBufferSizeEnablesPortBufferMarginEnablesPortSynchronicityEnablesPortSignalSizeEnablesPortBufferSizesPortBufferMarginsFunctionDeclFunctionTemplateSpecKindFunctionTemplateParamNamesFunctionTemplateParamKindsFunctionTemplateParamTypesFunctionTemplateParamValuesFunctionTemplateParamEnablesClassDeclClassTemplateSpecKindClassTemplateParamNamesClassTemplateParamKindsClassTemplateParamTypesClassTemplateParamValuesClassTemplateParamEnablesClassCtorDeclsClassCtorParamNamesClassCtorParamTypesClassCtorParamSerializedTypes[1 1]@C[32 1]@t21@exp_calc_float_lookupt22@../../exp_calc_float.hC[2 1]@t9@cb_input1t10@cb_output1C[2 1]@t38@adf::input_buffer< cfloat > & restrictt31@output_stream_cfloat * restrictC[2 1]@t42@{Q2{R{Tadf::input_buffer{1{t{Scfloat}}}}}}t38@{Q2{P{Toutput_stream{1{t{Scfloat}}}}}}C[2 1]@t5@inputt6@outputC[2 1]@l1@l0@C[2 1]@l1@l0@C[2 1]@l1@l0@C[2 1]@l0@l0@C[2 1]@l1@l0@C[2 1]@l0@l1@C[2 1]@nnC[2 1]@nnt159@template < unsigned int PHASE_INDEX > 
      | void exp_calc_float_lookup(adf::input_buffer< cfloat > & restrict cb_input1, output_stream_cfloat * restrict cb_output1)t8@implicitC[1 1]@t11@PHASE_INDEXC[1 1]@t7@nontypeC[1 1]@t12@unsigned intC[1 1]@nC[1 1]@l1@nne[0 1]@e[0 1]@e[0 1]@e[0 1]@e[0 1]@e[0 1]@e[0 1]@e[0 1]@e[0 1]@
      FunctionDeclTypeOptions=|
      | C[1 1]@t160@template < unsigned int PHASE_INDEX > 
      | void exp_calc_float_lookup(adf::input_buffer< cfloat > && restrict cb_input1, output_stream_cfloat * restrict cb_output1)
      FunctionDecl=|
      | template < unsigned int PHASE_INDEX > 
      | void exp_calc_float_lookup(adf::input_buffer< cfloat > && restrict cb_input1, output_stream_cfloat * restrict cb_output1)
  exp_calc_LUT23 : aieBasic/AIE Kernel  KernelAllAttrs=|  PortNames={'cb_input1'; 'cb_output1'}  PortSerializedTypes={'{Q2{R{Tadf::input_buffer{1{t{Scfloat}}}}}}'; '{Q2{P{Toutput_stream{1{t{Scfloat}}}}}}'}  PortWindowSizes={1.024000000000000000e+03, 0.000000000000000000e+00}  PortWindowMargins={0.000000000000000000e+00, 0.000000000000000000e+00}  PortSynchronicities={'sync', 'auto'}  PortSignalSizes={0.000000000000000000e+00; 1.024000000000000000e+03}  FunctionTemplateSpecKind=implicit  FunctionTemplateParamNames={'PHASE_INDEX'}  FunctionTemplateParamKinds={'nontype'}  FunctionTemplateParamTypes={'unsigned int'}  FunctionTemplateParamValues={'23'}  FunctionIndex=1  FunctionTabVisible=on  FunctionTemplateParamsVisible=on  FunctionDeclTypeOptions=|  FunctionDecl=|  FunctionTemplateParams={ 'PHASE_INDEX', 'unsigned int', '23' }  FunctionTemplateParamsEnables={'off', 'off', 'on'}  PortAttrs={ 'input', 'cb_input1', 'adf::input_buffer< cfloat > & restrict', '1024', '0', 'sync', ''; 'output', 'cb_output1', 'output_stream_cfloat * restrict', '', '', '', '1024' }  PortAttrsEnables={'off', 'off', 'off', 'on', 'off', 'off', 'off';'off', 'off', 'off', 'off', 'off', 'off', 'on'}  SampleTime=-1  KernelHeaderFile=exp_calc_float.h  KernelFunction=exp_calc_float_lookup  KernelSourceFile=exp_calc_float.cc  KernelSearchPaths={}  PreProcOptions={}  blockJsonConstraints=[]
      KernelAllAttrs=|
      | s[12;12;9;9;19;14;21;23;21;23;24;21;15;17;12;24;26;26;26;27;28;9;21;23;23;23;24;25;14;19;19;29]@FunctionNameDeclFileNamePortNamesPortTypesPortSerializedTypesPortDirectionsPortWindowSizeEnablesPortWindowMarginEnablesPortBufferSizeEnablesPortBufferMarginEnablesPortSynchronicityEnablesPortSignalSizeEnablesPortBufferSizesPortBufferMarginsFunctionDeclFunctionTemplateSpecKindFunctionTemplateParamNamesFunctionTemplateParamKindsFunctionTemplateParamTypesFunctionTemplateParamValuesFunctionTemplateParamEnablesClassDeclClassTemplateSpecKindClassTemplateParamNamesClassTemplateParamKindsClassTemplateParamTypesClassTemplateParamValuesClassTemplateParamEnablesClassCtorDeclsClassCtorParamNamesClassCtorParamTypesClassCtorParamSerializedTypes[1 1]@C[32 1]@t21@exp_calc_float_lookupt22@../../exp_calc_float.hC[2 1]@t9@cb_input1t10@cb_output1C[2 1]@t38@adf::input_buffer< cfloat > & restrictt31@output_stream_cfloat * restrictC[2 1]@t42@{Q2{R{Tadf::input_buffer{1{t{Scfloat}}}}}}t38@{Q2{P{Toutput_stream{1{t{Scfloat}}}}}}C[2 1]@t5@inputt6@outputC[2 1]@l1@l0@C[2 1]@l1@l0@C[2 1]@l1@l0@C[2 1]@l0@l0@C[2 1]@l1@l0@C[2 1]@l0@l1@C[2 1]@nnC[2 1]@nnt159@template < unsigned int PHASE_INDEX > 
      | void exp_calc_float_lookup(adf::input_buffer< cfloat > & restrict cb_input1, output_stream_cfloat * restrict cb_output1)t8@implicitC[1 1]@t11@PHASE_INDEXC[1 1]@t7@nontypeC[1 1]@t12@unsigned intC[1 1]@nC[1 1]@l1@nne[0 1]@e[0 1]@e[0 1]@e[0 1]@e[0 1]@e[0 1]@e[0 1]@e[0 1]@e[0 1]@
      FunctionDeclTypeOptions=|
      | C[1 1]@t160@template < unsigned int PHASE_INDEX > 
      | void exp_calc_float_lookup(adf::input_buffer< cfloat > && restrict cb_input1, output_stream_cfloat * restrict cb_output1)
      FunctionDecl=|
      | template < unsigned int PHASE_INDEX > 
      | void exp_calc_float_lookup(adf::input_buffer< cfloat > && restrict cb_input1, output_stream_cfloat * restrict cb_output1)
  exp_calc_LUT24 : aieBasic/AIE Kernel  KernelAllAttrs=|  PortNames={'cb_input1'; 'cb_output1'}  PortSerializedTypes={'{Q2{R{Tadf::input_buffer{1{t{Scfloat}}}}}}'; '{Q2{P{Toutput_stream{1{t{Scfloat}}}}}}'}  PortWindowSizes={1.024000000000000000e+03, 0.000000000000000000e+00}  PortWindowMargins={0.000000000000000000e+00, 0.000000000000000000e+00}  PortSynchronicities={'sync', 'auto'}  PortSignalSizes={0.000000000000000000e+00; 1.024000000000000000e+03}  FunctionTemplateSpecKind=implicit  FunctionTemplateParamNames={'PHASE_INDEX'}  FunctionTemplateParamKinds={'nontype'}  FunctionTemplateParamTypes={'unsigned int'}  FunctionTemplateParamValues={'24'}  FunctionIndex=1  FunctionTabVisible=on  FunctionTemplateParamsVisible=on  FunctionDeclTypeOptions=|  FunctionDecl=|  FunctionTemplateParams={ 'PHASE_INDEX', 'unsigned int', '24' }  FunctionTemplateParamsEnables={'off', 'off', 'on'}  PortAttrs={ 'input', 'cb_input1', 'adf::input_buffer< cfloat > & restrict', '1024', '0', 'sync', ''; 'output', 'cb_output1', 'output_stream_cfloat * restrict', '', '', '', '1024' }  PortAttrsEnables={'off', 'off', 'off', 'on', 'off', 'off', 'off';'off', 'off', 'off', 'off', 'off', 'off', 'on'}  SampleTime=-1  KernelHeaderFile=exp_calc_float.h  KernelFunction=exp_calc_float_lookup  KernelSourceFile=exp_calc_float.cc  KernelSearchPaths={}  PreProcOptions={}  blockJsonConstraints=[]
      KernelAllAttrs=|
      | s[12;12;9;9;19;14;21;23;21;23;24;21;15;17;12;24;26;26;26;27;28;9;21;23;23;23;24;25;14;19;19;29]@FunctionNameDeclFileNamePortNamesPortTypesPortSerializedTypesPortDirectionsPortWindowSizeEnablesPortWindowMarginEnablesPortBufferSizeEnablesPortBufferMarginEnablesPortSynchronicityEnablesPortSignalSizeEnablesPortBufferSizesPortBufferMarginsFunctionDeclFunctionTemplateSpecKindFunctionTemplateParamNamesFunctionTemplateParamKindsFunctionTemplateParamTypesFunctionTemplateParamValuesFunctionTemplateParamEnablesClassDeclClassTemplateSpecKindClassTemplateParamNamesClassTemplateParamKindsClassTemplateParamTypesClassTemplateParamValuesClassTemplateParamEnablesClassCtorDeclsClassCtorParamNamesClassCtorParamTypesClassCtorParamSerializedTypes[1 1]@C[32 1]@t21@exp_calc_float_lookupt22@../../exp_calc_float.hC[2 1]@t9@cb_input1t10@cb_output1C[2 1]@t38@adf::input_buffer< cfloat > & restrictt31@output_stream_cfloat * restrictC[2 1]@t42@{Q2{R{Tadf::input_buffer{1{t{Scfloat}}}}}}t38@{Q2{P{Toutput_stream{1{t{Scfloat}}}}}}C[2 1]@t5@inputt6@outputC[2 1]@l1@l0@C[2 1]@l1@l0@C[2 1]@l1@l0@C[2 1]@l0@l0@C[2 1]@l1@l0@C[2 1]@l0@l1@C[2 1]@nnC[2 1]@nnt159@template < unsigned int PHASE_INDEX > 
      | void exp_calc_float_lookup(adf::input_buffer< cfloat > & restrict cb_input1, output_stream_cfloat * restrict cb_output1)t8@implicitC[1 1]@t11@PHASE_INDEXC[1 1]@t7@nontypeC[1 1]@t12@unsigned intC[1 1]@nC[1 1]@l1@nne[0 1]@e[0 1]@e[0 1]@e[0 1]@e[0 1]@e[0 1]@e[0 1]@e[0 1]@e[0 1]@
      FunctionDeclTypeOptions=|
      | C[1 1]@t160@template < unsigned int PHASE_INDEX > 
      | void exp_calc_float_lookup(adf::input_buffer< cfloat > && restrict cb_input1, output_stream_cfloat * restrict cb_output1)
      FunctionDecl=|
      | template < unsigned int PHASE_INDEX > 
      | void exp_calc_float_lookup(adf::input_buffer< cfloat > && restrict cb_input1, output_stream_cfloat * restrict cb_output1)
  exp_calc_LUT25 : aieBasic/AIE Kernel  KernelAllAttrs=|  PortNames={'cb_input1'; 'cb_output1'}  PortSerializedTypes={'{Q2{R{Tadf::input_buffer{1{t{Scfloat}}}}}}'; '{Q2{P{Toutput_stream{1{t{Scfloat}}}}}}'}  PortWindowSizes={1.024000000000000000e+03, 0.000000000000000000e+00}  PortWindowMargins={0.000000000000000000e+00, 0.000000000000000000e+00}  PortSynchronicities={'sync', 'auto'}  PortSignalSizes={0.000000000000000000e+00; 1.024000000000000000e+03}  FunctionTemplateSpecKind=implicit  FunctionTemplateParamNames={'PHASE_INDEX'}  FunctionTemplateParamKinds={'nontype'}  FunctionTemplateParamTypes={'unsigned int'}  FunctionTemplateParamValues={'25'}  FunctionIndex=1  FunctionTabVisible=on  FunctionTemplateParamsVisible=on  FunctionDeclTypeOptions=|  FunctionDecl=|  FunctionTemplateParams={ 'PHASE_INDEX', 'unsigned int', '25' }  FunctionTemplateParamsEnables={'off', 'off', 'on'}  PortAttrs={ 'input', 'cb_input1', 'adf::input_buffer< cfloat > & restrict', '1024', '0', 'sync', ''; 'output', 'cb_output1', 'output_stream_cfloat * restrict', '', '', '', '1024' }  PortAttrsEnables={'off', 'off', 'off', 'on', 'off', 'off', 'off';'off', 'off', 'off', 'off', 'off', 'off', 'on'}  SampleTime=-1  KernelHeaderFile=exp_calc_float.h  KernelFunction=exp_calc_float_lookup  KernelSourceFile=exp_calc_float.cc  KernelSearchPaths={}  PreProcOptions={}  blockJsonConstraints=[]
      KernelAllAttrs=|
      | s[12;12;9;9;19;14;21;23;21;23;24;21;15;17;12;24;26;26;26;27;28;9;21;23;23;23;24;25;14;19;19;29]@FunctionNameDeclFileNamePortNamesPortTypesPortSerializedTypesPortDirectionsPortWindowSizeEnablesPortWindowMarginEnablesPortBufferSizeEnablesPortBufferMarginEnablesPortSynchronicityEnablesPortSignalSizeEnablesPortBufferSizesPortBufferMarginsFunctionDeclFunctionTemplateSpecKindFunctionTemplateParamNamesFunctionTemplateParamKindsFunctionTemplateParamTypesFunctionTemplateParamValuesFunctionTemplateParamEnablesClassDeclClassTemplateSpecKindClassTemplateParamNamesClassTemplateParamKindsClassTemplateParamTypesClassTemplateParamValuesClassTemplateParamEnablesClassCtorDeclsClassCtorParamNamesClassCtorParamTypesClassCtorParamSerializedTypes[1 1]@C[32 1]@t21@exp_calc_float_lookupt22@../../exp_calc_float.hC[2 1]@t9@cb_input1t10@cb_output1C[2 1]@t38@adf::input_buffer< cfloat > & restrictt31@output_stream_cfloat * restrictC[2 1]@t42@{Q2{R{Tadf::input_buffer{1{t{Scfloat}}}}}}t38@{Q2{P{Toutput_stream{1{t{Scfloat}}}}}}C[2 1]@t5@inputt6@outputC[2 1]@l1@l0@C[2 1]@l1@l0@C[2 1]@l1@l0@C[2 1]@l0@l0@C[2 1]@l1@l0@C[2 1]@l0@l1@C[2 1]@nnC[2 1]@nnt159@template < unsigned int PHASE_INDEX > 
      | void exp_calc_float_lookup(adf::input_buffer< cfloat > & restrict cb_input1, output_stream_cfloat * restrict cb_output1)t8@implicitC[1 1]@t11@PHASE_INDEXC[1 1]@t7@nontypeC[1 1]@t12@unsigned intC[1 1]@nC[1 1]@l1@nne[0 1]@e[0 1]@e[0 1]@e[0 1]@e[0 1]@e[0 1]@e[0 1]@e[0 1]@e[0 1]@
      FunctionDeclTypeOptions=|
      | C[1 1]@t160@template < unsigned int PHASE_INDEX > 
      | void exp_calc_float_lookup(adf::input_buffer< cfloat > && restrict cb_input1, output_stream_cfloat * restrict cb_output1)
      FunctionDecl=|
      | template < unsigned int PHASE_INDEX > 
      | void exp_calc_float_lookup(adf::input_buffer< cfloat > && restrict cb_input1, output_stream_cfloat * restrict cb_output1)
  exp_calc_LUT26 : aieBasic/AIE Kernel  KernelAllAttrs=|  PortNames={'cb_input1'; 'cb_output1'}  PortSerializedTypes={'{Q2{R{Tadf::input_buffer{1{t{Scfloat}}}}}}'; '{Q2{P{Toutput_stream{1{t{Scfloat}}}}}}'}  PortWindowSizes={1.024000000000000000e+03, 0.000000000000000000e+00}  PortWindowMargins={0.000000000000000000e+00, 0.000000000000000000e+00}  PortSynchronicities={'sync', 'auto'}  PortSignalSizes={0.000000000000000000e+00; 1.024000000000000000e+03}  FunctionTemplateSpecKind=implicit  FunctionTemplateParamNames={'PHASE_INDEX'}  FunctionTemplateParamKinds={'nontype'}  FunctionTemplateParamTypes={'unsigned int'}  FunctionTemplateParamValues={'26'}  FunctionIndex=1  FunctionTabVisible=on  FunctionTemplateParamsVisible=on  FunctionDeclTypeOptions=|  FunctionDecl=|  FunctionTemplateParams={ 'PHASE_INDEX', 'unsigned int', '26' }  FunctionTemplateParamsEnables={'off', 'off', 'on'}  PortAttrs={ 'input', 'cb_input1', 'adf::input_buffer< cfloat > & restrict', '1024', '0', 'sync', ''; 'output', 'cb_output1', 'output_stream_cfloat * restrict', '', '', '', '1024' }  PortAttrsEnables={'off', 'off', 'off', 'on', 'off', 'off', 'off';'off', 'off', 'off', 'off', 'off', 'off', 'on'}  SampleTime=-1  KernelHeaderFile=exp_calc_float.h  KernelFunction=exp_calc_float_lookup  KernelSourceFile=exp_calc_float.cc  KernelSearchPaths={}  PreProcOptions={}  blockJsonConstraints=[]
      KernelAllAttrs=|
      | s[12;12;9;9;19;14;21;23;21;23;24;21;15;17;12;24;26;26;26;27;28;9;21;23;23;23;24;25;14;19;19;29]@FunctionNameDeclFileNamePortNamesPortTypesPortSerializedTypesPortDirectionsPortWindowSizeEnablesPortWindowMarginEnablesPortBufferSizeEnablesPortBufferMarginEnablesPortSynchronicityEnablesPortSignalSizeEnablesPortBufferSizesPortBufferMarginsFunctionDeclFunctionTemplateSpecKindFunctionTemplateParamNamesFunctionTemplateParamKindsFunctionTemplateParamTypesFunctionTemplateParamValuesFunctionTemplateParamEnablesClassDeclClassTemplateSpecKindClassTemplateParamNamesClassTemplateParamKindsClassTemplateParamTypesClassTemplateParamValuesClassTemplateParamEnablesClassCtorDeclsClassCtorParamNamesClassCtorParamTypesClassCtorParamSerializedTypes[1 1]@C[32 1]@t21@exp_calc_float_lookupt22@../../exp_calc_float.hC[2 1]@t9@cb_input1t10@cb_output1C[2 1]@t38@adf::input_buffer< cfloat > & restrictt31@output_stream_cfloat * restrictC[2 1]@t42@{Q2{R{Tadf::input_buffer{1{t{Scfloat}}}}}}t38@{Q2{P{Toutput_stream{1{t{Scfloat}}}}}}C[2 1]@t5@inputt6@outputC[2 1]@l1@l0@C[2 1]@l1@l0@C[2 1]@l1@l0@C[2 1]@l0@l0@C[2 1]@l1@l0@C[2 1]@l0@l1@C[2 1]@nnC[2 1]@nnt159@template < unsigned int PHASE_INDEX > 
      | void exp_calc_float_lookup(adf::input_buffer< cfloat > & restrict cb_input1, output_stream_cfloat * restrict cb_output1)t8@implicitC[1 1]@t11@PHASE_INDEXC[1 1]@t7@nontypeC[1 1]@t12@unsigned intC[1 1]@nC[1 1]@l1@nne[0 1]@e[0 1]@e[0 1]@e[0 1]@e[0 1]@e[0 1]@e[0 1]@e[0 1]@e[0 1]@
      FunctionDeclTypeOptions=|
      | C[1 1]@t160@template < unsigned int PHASE_INDEX > 
      | void exp_calc_float_lookup(adf::input_buffer< cfloat > && restrict cb_input1, output_stream_cfloat * restrict cb_output1)
      FunctionDecl=|
      | template < unsigned int PHASE_INDEX > 
      | void exp_calc_float_lookup(adf::input_buffer< cfloat > && restrict cb_input1, output_stream_cfloat * restrict cb_output1)
  exp_calc_LUT27 : aieBasic/AIE Kernel  KernelAllAttrs=|  PortNames={'cb_input1'; 'cb_output1'}  PortSerializedTypes={'{Q2{R{Tadf::input_buffer{1{t{Scfloat}}}}}}'; '{Q2{P{Toutput_stream{1{t{Scfloat}}}}}}'}  PortWindowSizes={1.024000000000000000e+03, 0.000000000000000000e+00}  PortWindowMargins={0.000000000000000000e+00, 0.000000000000000000e+00}  PortSynchronicities={'sync', 'auto'}  PortSignalSizes={0.000000000000000000e+00; 1.024000000000000000e+03}  FunctionTemplateSpecKind=implicit  FunctionTemplateParamNames={'PHASE_INDEX'}  FunctionTemplateParamKinds={'nontype'}  FunctionTemplateParamTypes={'unsigned int'}  FunctionTemplateParamValues={'27'}  FunctionIndex=1  FunctionTabVisible=on  FunctionTemplateParamsVisible=on  FunctionDeclTypeOptions=|  FunctionDecl=|  FunctionTemplateParams={ 'PHASE_INDEX', 'unsigned int', '27' }  FunctionTemplateParamsEnables={'off', 'off', 'on'}  PortAttrs={ 'input', 'cb_input1', 'adf::input_buffer< cfloat > & restrict', '1024', '0', 'sync', ''; 'output', 'cb_output1', 'output_stream_cfloat * restrict', '', '', '', '1024' }  PortAttrsEnables={'off', 'off', 'off', 'on', 'off', 'off', 'off';'off', 'off', 'off', 'off', 'off', 'off', 'on'}  SampleTime=-1  KernelHeaderFile=exp_calc_float.h  KernelFunction=exp_calc_float_lookup  KernelSourceFile=exp_calc_float.cc  KernelSearchPaths={}  PreProcOptions={}  blockJsonConstraints=[]
      KernelAllAttrs=|
      | s[12;12;9;9;19;14;21;23;21;23;24;21;15;17;12;24;26;26;26;27;28;9;21;23;23;23;24;25;14;19;19;29]@FunctionNameDeclFileNamePortNamesPortTypesPortSerializedTypesPortDirectionsPortWindowSizeEnablesPortWindowMarginEnablesPortBufferSizeEnablesPortBufferMarginEnablesPortSynchronicityEnablesPortSignalSizeEnablesPortBufferSizesPortBufferMarginsFunctionDeclFunctionTemplateSpecKindFunctionTemplateParamNamesFunctionTemplateParamKindsFunctionTemplateParamTypesFunctionTemplateParamValuesFunctionTemplateParamEnablesClassDeclClassTemplateSpecKindClassTemplateParamNamesClassTemplateParamKindsClassTemplateParamTypesClassTemplateParamValuesClassTemplateParamEnablesClassCtorDeclsClassCtorParamNamesClassCtorParamTypesClassCtorParamSerializedTypes[1 1]@C[32 1]@t21@exp_calc_float_lookupt22@../../exp_calc_float.hC[2 1]@t9@cb_input1t10@cb_output1C[2 1]@t38@adf::input_buffer< cfloat > & restrictt31@output_stream_cfloat * restrictC[2 1]@t42@{Q2{R{Tadf::input_buffer{1{t{Scfloat}}}}}}t38@{Q2{P{Toutput_stream{1{t{Scfloat}}}}}}C[2 1]@t5@inputt6@outputC[2 1]@l1@l0@C[2 1]@l1@l0@C[2 1]@l1@l0@C[2 1]@l0@l0@C[2 1]@l1@l0@C[2 1]@l0@l1@C[2 1]@nnC[2 1]@nnt159@template < unsigned int PHASE_INDEX > 
      | void exp_calc_float_lookup(adf::input_buffer< cfloat > & restrict cb_input1, output_stream_cfloat * restrict cb_output1)t8@implicitC[1 1]@t11@PHASE_INDEXC[1 1]@t7@nontypeC[1 1]@t12@unsigned intC[1 1]@nC[1 1]@l1@nne[0 1]@e[0 1]@e[0 1]@e[0 1]@e[0 1]@e[0 1]@e[0 1]@e[0 1]@e[0 1]@
      FunctionDeclTypeOptions=|
      | C[1 1]@t160@template < unsigned int PHASE_INDEX > 
      | void exp_calc_float_lookup(adf::input_buffer< cfloat > && restrict cb_input1, output_stream_cfloat * restrict cb_output1)
      FunctionDecl=|
      | template < unsigned int PHASE_INDEX > 
      | void exp_calc_float_lookup(adf::input_buffer< cfloat > && restrict cb_input1, output_stream_cfloat * restrict cb_output1)
  exp_calc_LUT28 : aieBasic/AIE Kernel  KernelAllAttrs=|  PortNames={'cb_input1'; 'cb_output1'}  PortSerializedTypes={'{Q2{R{Tadf::input_buffer{1{t{Scfloat}}}}}}'; '{Q2{P{Toutput_stream{1{t{Scfloat}}}}}}'}  PortWindowSizes={1.024000000000000000e+03, 0.000000000000000000e+00}  PortWindowMargins={0.000000000000000000e+00, 0.000000000000000000e+00}  PortSynchronicities={'sync', 'auto'}  PortSignalSizes={0.000000000000000000e+00; 1.024000000000000000e+03}  FunctionTemplateSpecKind=implicit  FunctionTemplateParamNames={'PHASE_INDEX'}  FunctionTemplateParamKinds={'nontype'}  FunctionTemplateParamTypes={'unsigned int'}  FunctionTemplateParamValues={'28'}  FunctionIndex=1  FunctionTabVisible=on  FunctionTemplateParamsVisible=on  FunctionDeclTypeOptions=|  FunctionDecl=|  FunctionTemplateParams={ 'PHASE_INDEX', 'unsigned int', '28' }  FunctionTemplateParamsEnables={'off', 'off', 'on'}  PortAttrs={ 'input', 'cb_input1', 'adf::input_buffer< cfloat > & restrict', '1024', '0', 'sync', ''; 'output', 'cb_output1', 'output_stream_cfloat * restrict', '', '', '', '1024' }  PortAttrsEnables={'off', 'off', 'off', 'on', 'off', 'off', 'off';'off', 'off', 'off', 'off', 'off', 'off', 'on'}  SampleTime=-1  KernelHeaderFile=exp_calc_float.h  KernelFunction=exp_calc_float_lookup  KernelSourceFile=exp_calc_float.cc  KernelSearchPaths={}  PreProcOptions={}  blockJsonConstraints=[]
      KernelAllAttrs=|
      | s[12;12;9;9;19;14;21;23;21;23;24;21;15;17;12;24;26;26;26;27;28;9;21;23;23;23;24;25;14;19;19;29]@FunctionNameDeclFileNamePortNamesPortTypesPortSerializedTypesPortDirectionsPortWindowSizeEnablesPortWindowMarginEnablesPortBufferSizeEnablesPortBufferMarginEnablesPortSynchronicityEnablesPortSignalSizeEnablesPortBufferSizesPortBufferMarginsFunctionDeclFunctionTemplateSpecKindFunctionTemplateParamNamesFunctionTemplateParamKindsFunctionTemplateParamTypesFunctionTemplateParamValuesFunctionTemplateParamEnablesClassDeclClassTemplateSpecKindClassTemplateParamNamesClassTemplateParamKindsClassTemplateParamTypesClassTemplateParamValuesClassTemplateParamEnablesClassCtorDeclsClassCtorParamNamesClassCtorParamTypesClassCtorParamSerializedTypes[1 1]@C[32 1]@t21@exp_calc_float_lookupt22@../../exp_calc_float.hC[2 1]@t9@cb_input1t10@cb_output1C[2 1]@t38@adf::input_buffer< cfloat > & restrictt31@output_stream_cfloat * restrictC[2 1]@t42@{Q2{R{Tadf::input_buffer{1{t{Scfloat}}}}}}t38@{Q2{P{Toutput_stream{1{t{Scfloat}}}}}}C[2 1]@t5@inputt6@outputC[2 1]@l1@l0@C[2 1]@l1@l0@C[2 1]@l1@l0@C[2 1]@l0@l0@C[2 1]@l1@l0@C[2 1]@l0@l1@C[2 1]@nnC[2 1]@nnt159@template < unsigned int PHASE_INDEX > 
      | void exp_calc_float_lookup(adf::input_buffer< cfloat > & restrict cb_input1, output_stream_cfloat * restrict cb_output1)t8@implicitC[1 1]@t11@PHASE_INDEXC[1 1]@t7@nontypeC[1 1]@t12@unsigned intC[1 1]@nC[1 1]@l1@nne[0 1]@e[0 1]@e[0 1]@e[0 1]@e[0 1]@e[0 1]@e[0 1]@e[0 1]@e[0 1]@
      FunctionDeclTypeOptions=|
      | C[1 1]@t160@template < unsigned int PHASE_INDEX > 
      | void exp_calc_float_lookup(adf::input_buffer< cfloat > && restrict cb_input1, output_stream_cfloat * restrict cb_output1)
      FunctionDecl=|
      | template < unsigned int PHASE_INDEX > 
      | void exp_calc_float_lookup(adf::input_buffer< cfloat > && restrict cb_input1, output_stream_cfloat * restrict cb_output1)
  exp_calc_LUT29 : aieBasic/AIE Kernel  KernelAllAttrs=|  PortNames={'cb_input1'; 'cb_output1'}  PortSerializedTypes={'{Q2{R{Tadf::input_buffer{1{t{Scfloat}}}}}}'; '{Q2{P{Toutput_stream{1{t{Scfloat}}}}}}'}  PortWindowSizes={1.024000000000000000e+03, 0.000000000000000000e+00}  PortWindowMargins={0.000000000000000000e+00, 0.000000000000000000e+00}  PortSynchronicities={'sync', 'auto'}  PortSignalSizes={0.000000000000000000e+00; 1.024000000000000000e+03}  FunctionTemplateSpecKind=implicit  FunctionTemplateParamNames={'PHASE_INDEX'}  FunctionTemplateParamKinds={'nontype'}  FunctionTemplateParamTypes={'unsigned int'}  FunctionTemplateParamValues={'29'}  FunctionIndex=1  FunctionTabVisible=on  FunctionTemplateParamsVisible=on  FunctionDeclTypeOptions=|  FunctionDecl=|  FunctionTemplateParams={ 'PHASE_INDEX', 'unsigned int', '29' }  FunctionTemplateParamsEnables={'off', 'off', 'on'}  PortAttrs={ 'input', 'cb_input1', 'adf::input_buffer< cfloat > & restrict', '1024', '0', 'sync', ''; 'output', 'cb_output1', 'output_stream_cfloat * restrict', '', '', '', '1024' }  PortAttrsEnables={'off', 'off', 'off', 'on', 'off', 'off', 'off';'off', 'off', 'off', 'off', 'off', 'off', 'on'}  SampleTime=-1  KernelHeaderFile=exp_calc_float.h  KernelFunction=exp_calc_float_lookup  KernelSourceFile=exp_calc_float.cc  KernelSearchPaths={}  PreProcOptions={}  blockJsonConstraints=[]
      KernelAllAttrs=|
      | s[12;12;9;9;19;14;21;23;21;23;24;21;15;17;12;24;26;26;26;27;28;9;21;23;23;23;24;25;14;19;19;29]@FunctionNameDeclFileNamePortNamesPortTypesPortSerializedTypesPortDirectionsPortWindowSizeEnablesPortWindowMarginEnablesPortBufferSizeEnablesPortBufferMarginEnablesPortSynchronicityEnablesPortSignalSizeEnablesPortBufferSizesPortBufferMarginsFunctionDeclFunctionTemplateSpecKindFunctionTemplateParamNamesFunctionTemplateParamKindsFunctionTemplateParamTypesFunctionTemplateParamValuesFunctionTemplateParamEnablesClassDeclClassTemplateSpecKindClassTemplateParamNamesClassTemplateParamKindsClassTemplateParamTypesClassTemplateParamValuesClassTemplateParamEnablesClassCtorDeclsClassCtorParamNamesClassCtorParamTypesClassCtorParamSerializedTypes[1 1]@C[32 1]@t21@exp_calc_float_lookupt22@../../exp_calc_float.hC[2 1]@t9@cb_input1t10@cb_output1C[2 1]@t38@adf::input_buffer< cfloat > & restrictt31@output_stream_cfloat * restrictC[2 1]@t42@{Q2{R{Tadf::input_buffer{1{t{Scfloat}}}}}}t38@{Q2{P{Toutput_stream{1{t{Scfloat}}}}}}C[2 1]@t5@inputt6@outputC[2 1]@l1@l0@C[2 1]@l1@l0@C[2 1]@l1@l0@C[2 1]@l0@l0@C[2 1]@l1@l0@C[2 1]@l0@l1@C[2 1]@nnC[2 1]@nnt159@template < unsigned int PHASE_INDEX > 
      | void exp_calc_float_lookup(adf::input_buffer< cfloat > & restrict cb_input1, output_stream_cfloat * restrict cb_output1)t8@implicitC[1 1]@t11@PHASE_INDEXC[1 1]@t7@nontypeC[1 1]@t12@unsigned intC[1 1]@nC[1 1]@l1@nne[0 1]@e[0 1]@e[0 1]@e[0 1]@e[0 1]@e[0 1]@e[0 1]@e[0 1]@e[0 1]@
      FunctionDeclTypeOptions=|
      | C[1 1]@t160@template < unsigned int PHASE_INDEX > 
      | void exp_calc_float_lookup(adf::input_buffer< cfloat > && restrict cb_input1, output_stream_cfloat * restrict cb_output1)
      FunctionDecl=|
      | template < unsigned int PHASE_INDEX > 
      | void exp_calc_float_lookup(adf::input_buffer< cfloat > && restrict cb_input1, output_stream_cfloat * restrict cb_output1)
  exp_calc_LUT3 : aieBasic/AIE Kernel  KernelAllAttrs=|  PortNames={'cb_input1'; 'cb_output1'}  PortSerializedTypes={'{Q2{R{Tadf::input_buffer{1{t{Scfloat}}}}}}'; '{Q2{P{Toutput_stream{1{t{Scfloat}}}}}}'}  PortWindowSizes={1.024000000000000000e+03, 0.000000000000000000e+00}  PortWindowMargins={0.000000000000000000e+00, 0.000000000000000000e+00}  PortSynchronicities={'sync', 'auto'}  PortSignalSizes={0.000000000000000000e+00; 1.024000000000000000e+03}  FunctionTemplateSpecKind=implicit  FunctionTemplateParamNames={'PHASE_INDEX'}  FunctionTemplateParamKinds={'nontype'}  FunctionTemplateParamTypes={'unsigned int'}  FunctionTemplateParamValues={'3'}  FunctionIndex=1  FunctionTabVisible=on  FunctionTemplateParamsVisible=on  FunctionDeclTypeOptions=|  FunctionDecl=|  FunctionTemplateParams={ 'PHASE_INDEX', 'unsigned int', '3' }  FunctionTemplateParamsEnables={'off', 'off', 'on'}  PortAttrs={ 'input', 'cb_input1', 'adf::input_buffer< cfloat > & restrict', '1024', '0', 'sync', ''; 'output', 'cb_output1', 'output_stream_cfloat * restrict', '', '', '', '1024' }  PortAttrsEnables={'off', 'off', 'off', 'on', 'off', 'off', 'off';'off', 'off', 'off', 'off', 'off', 'off', 'on'}  SampleTime=-1  KernelHeaderFile=exp_calc_float.h  KernelFunction=exp_calc_float_lookup  KernelSourceFile=exp_calc_float.cc  KernelSearchPaths={}  PreProcOptions={}  blockJsonConstraints=[]
      KernelAllAttrs=|
      | s[12;12;9;9;19;14;21;23;21;23;24;21;15;17;12;24;26;26;26;27;28;9;21;23;23;23;24;25;14;19;19;29]@FunctionNameDeclFileNamePortNamesPortTypesPortSerializedTypesPortDirectionsPortWindowSizeEnablesPortWindowMarginEnablesPortBufferSizeEnablesPortBufferMarginEnablesPortSynchronicityEnablesPortSignalSizeEnablesPortBufferSizesPortBufferMarginsFunctionDeclFunctionTemplateSpecKindFunctionTemplateParamNamesFunctionTemplateParamKindsFunctionTemplateParamTypesFunctionTemplateParamValuesFunctionTemplateParamEnablesClassDeclClassTemplateSpecKindClassTemplateParamNamesClassTemplateParamKindsClassTemplateParamTypesClassTemplateParamValuesClassTemplateParamEnablesClassCtorDeclsClassCtorParamNamesClassCtorParamTypesClassCtorParamSerializedTypes[1 1]@C[32 1]@t21@exp_calc_float_lookupt22@../../exp_calc_float.hC[2 1]@t9@cb_input1t10@cb_output1C[2 1]@t38@adf::input_buffer< cfloat > & restrictt31@output_stream_cfloat * restrictC[2 1]@t42@{Q2{R{Tadf::input_buffer{1{t{Scfloat}}}}}}t38@{Q2{P{Toutput_stream{1{t{Scfloat}}}}}}C[2 1]@t5@inputt6@outputC[2 1]@l1@l0@C[2 1]@l1@l0@C[2 1]@l1@l0@C[2 1]@l0@l0@C[2 1]@l1@l0@C[2 1]@l0@l1@C[2 1]@nnC[2 1]@nnt159@template < unsigned int PHASE_INDEX > 
      | void exp_calc_float_lookup(adf::input_buffer< cfloat > & restrict cb_input1, output_stream_cfloat * restrict cb_output1)t8@implicitC[1 1]@t11@PHASE_INDEXC[1 1]@t7@nontypeC[1 1]@t12@unsigned intC[1 1]@nC[1 1]@l1@nne[0 1]@e[0 1]@e[0 1]@e[0 1]@e[0 1]@e[0 1]@e[0 1]@e[0 1]@e[0 1]@
      FunctionDeclTypeOptions=|
      | C[1 1]@t160@template < unsigned int PHASE_INDEX > 
      | void exp_calc_float_lookup(adf::input_buffer< cfloat > && restrict cb_input1, output_stream_cfloat * restrict cb_output1)
      FunctionDecl=|
      | template < unsigned int PHASE_INDEX > 
      | void exp_calc_float_lookup(adf::input_buffer< cfloat > && restrict cb_input1, output_stream_cfloat * restrict cb_output1)
  exp_calc_LUT30 : aieBasic/AIE Kernel  KernelAllAttrs=|  PortNames={'cb_input1'; 'cb_output1'}  PortSerializedTypes={'{Q2{R{Tadf::input_buffer{1{t{Scfloat}}}}}}'; '{Q2{P{Toutput_stream{1{t{Scfloat}}}}}}'}  PortWindowSizes={1.024000000000000000e+03, 0.000000000000000000e+00}  PortWindowMargins={0.000000000000000000e+00, 0.000000000000000000e+00}  PortSynchronicities={'sync', 'auto'}  PortSignalSizes={0.000000000000000000e+00; 1.024000000000000000e+03}  FunctionTemplateSpecKind=implicit  FunctionTemplateParamNames={'PHASE_INDEX'}  FunctionTemplateParamKinds={'nontype'}  FunctionTemplateParamTypes={'unsigned int'}  FunctionTemplateParamValues={'30'}  FunctionIndex=1  FunctionTabVisible=on  FunctionTemplateParamsVisible=on  FunctionDeclTypeOptions=|  FunctionDecl=|  FunctionTemplateParams={ 'PHASE_INDEX', 'unsigned int', '30' }  FunctionTemplateParamsEnables={'off', 'off', 'on'}  PortAttrs={ 'input', 'cb_input1', 'adf::input_buffer< cfloat > & restrict', '1024', '0', 'sync', ''; 'output', 'cb_output1', 'output_stream_cfloat * restrict', '', '', '', '1024' }  PortAttrsEnables={'off', 'off', 'off', 'on', 'off', 'off', 'off';'off', 'off', 'off', 'off', 'off', 'off', 'on'}  SampleTime=-1  KernelHeaderFile=exp_calc_float.h  KernelFunction=exp_calc_float_lookup  KernelSourceFile=exp_calc_float.cc  KernelSearchPaths={}  PreProcOptions={}  blockJsonConstraints=[]
      KernelAllAttrs=|
      | s[12;12;9;9;19;14;21;23;21;23;24;21;15;17;12;24;26;26;26;27;28;9;21;23;23;23;24;25;14;19;19;29]@FunctionNameDeclFileNamePortNamesPortTypesPortSerializedTypesPortDirectionsPortWindowSizeEnablesPortWindowMarginEnablesPortBufferSizeEnablesPortBufferMarginEnablesPortSynchronicityEnablesPortSignalSizeEnablesPortBufferSizesPortBufferMarginsFunctionDeclFunctionTemplateSpecKindFunctionTemplateParamNamesFunctionTemplateParamKindsFunctionTemplateParamTypesFunctionTemplateParamValuesFunctionTemplateParamEnablesClassDeclClassTemplateSpecKindClassTemplateParamNamesClassTemplateParamKindsClassTemplateParamTypesClassTemplateParamValuesClassTemplateParamEnablesClassCtorDeclsClassCtorParamNamesClassCtorParamTypesClassCtorParamSerializedTypes[1 1]@C[32 1]@t21@exp_calc_float_lookupt22@../../exp_calc_float.hC[2 1]@t9@cb_input1t10@cb_output1C[2 1]@t38@adf::input_buffer< cfloat > & restrictt31@output_stream_cfloat * restrictC[2 1]@t42@{Q2{R{Tadf::input_buffer{1{t{Scfloat}}}}}}t38@{Q2{P{Toutput_stream{1{t{Scfloat}}}}}}C[2 1]@t5@inputt6@outputC[2 1]@l1@l0@C[2 1]@l1@l0@C[2 1]@l1@l0@C[2 1]@l0@l0@C[2 1]@l1@l0@C[2 1]@l0@l1@C[2 1]@nnC[2 1]@nnt159@template < unsigned int PHASE_INDEX > 
      | void exp_calc_float_lookup(adf::input_buffer< cfloat > & restrict cb_input1, output_stream_cfloat * restrict cb_output1)t8@implicitC[1 1]@t11@PHASE_INDEXC[1 1]@t7@nontypeC[1 1]@t12@unsigned intC[1 1]@nC[1 1]@l1@nne[0 1]@e[0 1]@e[0 1]@e[0 1]@e[0 1]@e[0 1]@e[0 1]@e[0 1]@e[0 1]@
      FunctionDeclTypeOptions=|
      | C[1 1]@t160@template < unsigned int PHASE_INDEX > 
      | void exp_calc_float_lookup(adf::input_buffer< cfloat > && restrict cb_input1, output_stream_cfloat * restrict cb_output1)
      FunctionDecl=|
      | template < unsigned int PHASE_INDEX > 
      | void exp_calc_float_lookup(adf::input_buffer< cfloat > && restrict cb_input1, output_stream_cfloat * restrict cb_output1)
  exp_calc_LUT31 : aieBasic/AIE Kernel  KernelAllAttrs=|  PortNames={'cb_input1'; 'cb_output1'}  PortSerializedTypes={'{Q2{R{Tadf::input_buffer{1{t{Scfloat}}}}}}'; '{Q2{P{Toutput_stream{1{t{Scfloat}}}}}}'}  PortWindowSizes={1.024000000000000000e+03, 0.000000000000000000e+00}  PortWindowMargins={0.000000000000000000e+00, 0.000000000000000000e+00}  PortSynchronicities={'sync', 'auto'}  PortSignalSizes={0.000000000000000000e+00; 1.024000000000000000e+03}  FunctionTemplateSpecKind=implicit  FunctionTemplateParamNames={'PHASE_INDEX'}  FunctionTemplateParamKinds={'nontype'}  FunctionTemplateParamTypes={'unsigned int'}  FunctionTemplateParamValues={'31'}  FunctionIndex=1  FunctionTabVisible=on  FunctionTemplateParamsVisible=on  FunctionDeclTypeOptions=|  FunctionDecl=|  FunctionTemplateParams={ 'PHASE_INDEX', 'unsigned int', '31' }  FunctionTemplateParamsEnables={'off', 'off', 'on'}  PortAttrs={ 'input', 'cb_input1', 'adf::input_buffer< cfloat > & restrict', '1024', '0', 'sync', ''; 'output', 'cb_output1', 'output_stream_cfloat * restrict', '', '', '', '1024' }  PortAttrsEnables={'off', 'off', 'off', 'on', 'off', 'off', 'off';'off', 'off', 'off', 'off', 'off', 'off', 'on'}  SampleTime=-1  KernelHeaderFile=exp_calc_float.h  KernelFunction=exp_calc_float_lookup  KernelSourceFile=exp_calc_float.cc  KernelSearchPaths={}  PreProcOptions={}  blockJsonConstraints=[]
      KernelAllAttrs=|
      | s[12;12;9;9;19;14;21;23;21;23;24;21;15;17;12;24;26;26;26;27;28;9;21;23;23;23;24;25;14;19;19;29]@FunctionNameDeclFileNamePortNamesPortTypesPortSerializedTypesPortDirectionsPortWindowSizeEnablesPortWindowMarginEnablesPortBufferSizeEnablesPortBufferMarginEnablesPortSynchronicityEnablesPortSignalSizeEnablesPortBufferSizesPortBufferMarginsFunctionDeclFunctionTemplateSpecKindFunctionTemplateParamNamesFunctionTemplateParamKindsFunctionTemplateParamTypesFunctionTemplateParamValuesFunctionTemplateParamEnablesClassDeclClassTemplateSpecKindClassTemplateParamNamesClassTemplateParamKindsClassTemplateParamTypesClassTemplateParamValuesClassTemplateParamEnablesClassCtorDeclsClassCtorParamNamesClassCtorParamTypesClassCtorParamSerializedTypes[1 1]@C[32 1]@t21@exp_calc_float_lookupt22@../../exp_calc_float.hC[2 1]@t9@cb_input1t10@cb_output1C[2 1]@t38@adf::input_buffer< cfloat > & restrictt31@output_stream_cfloat * restrictC[2 1]@t42@{Q2{R{Tadf::input_buffer{1{t{Scfloat}}}}}}t38@{Q2{P{Toutput_stream{1{t{Scfloat}}}}}}C[2 1]@t5@inputt6@outputC[2 1]@l1@l0@C[2 1]@l1@l0@C[2 1]@l1@l0@C[2 1]@l0@l0@C[2 1]@l1@l0@C[2 1]@l0@l1@C[2 1]@nnC[2 1]@nnt159@template < unsigned int PHASE_INDEX > 
      | void exp_calc_float_lookup(adf::input_buffer< cfloat > & restrict cb_input1, output_stream_cfloat * restrict cb_output1)t8@implicitC[1 1]@t11@PHASE_INDEXC[1 1]@t7@nontypeC[1 1]@t12@unsigned intC[1 1]@nC[1 1]@l1@nne[0 1]@e[0 1]@e[0 1]@e[0 1]@e[0 1]@e[0 1]@e[0 1]@e[0 1]@e[0 1]@
      FunctionDeclTypeOptions=|
      | C[1 1]@t160@template < unsigned int PHASE_INDEX > 
      | void exp_calc_float_lookup(adf::input_buffer< cfloat > && restrict cb_input1, output_stream_cfloat * restrict cb_output1)
      FunctionDecl=|
      | template < unsigned int PHASE_INDEX > 
      | void exp_calc_float_lookup(adf::input_buffer< cfloat > && restrict cb_input1, output_stream_cfloat * restrict cb_output1)
  exp_calc_LUT4 : aieBasic/AIE Kernel  KernelAllAttrs=|  PortNames={'cb_input1'; 'cb_output1'}  PortSerializedTypes={'{Q2{R{Tadf::input_buffer{1{t{Scfloat}}}}}}'; '{Q2{P{Toutput_stream{1{t{Scfloat}}}}}}'}  PortWindowSizes={1.024000000000000000e+03, 0.000000000000000000e+00}  PortWindowMargins={0.000000000000000000e+00, 0.000000000000000000e+00}  PortSynchronicities={'sync', 'auto'}  PortSignalSizes={0.000000000000000000e+00; 1.024000000000000000e+03}  FunctionTemplateSpecKind=implicit  FunctionTemplateParamNames={'PHASE_INDEX'}  FunctionTemplateParamKinds={'nontype'}  FunctionTemplateParamTypes={'unsigned int'}  FunctionTemplateParamValues={'4'}  FunctionIndex=1  FunctionTabVisible=on  FunctionTemplateParamsVisible=on  FunctionDeclTypeOptions=|  FunctionDecl=|  FunctionTemplateParams={ 'PHASE_INDEX', 'unsigned int', '4' }  FunctionTemplateParamsEnables={'off', 'off', 'on'}  PortAttrs={ 'input', 'cb_input1', 'adf::input_buffer< cfloat > & restrict', '1024', '0', 'sync', ''; 'output', 'cb_output1', 'output_stream_cfloat * restrict', '', '', '', '1024' }  PortAttrsEnables={'off', 'off', 'off', 'on', 'off', 'off', 'off';'off', 'off', 'off', 'off', 'off', 'off', 'on'}  SampleTime=-1  KernelHeaderFile=exp_calc_float.h  KernelFunction=exp_calc_float_lookup  KernelSourceFile=exp_calc_float.cc  KernelSearchPaths={}  PreProcOptions={}  blockJsonConstraints=[]
      KernelAllAttrs=|
      | s[12;12;9;9;19;14;21;23;21;23;24;21;15;17;12;24;26;26;26;27;28;9;21;23;23;23;24;25;14;19;19;29]@FunctionNameDeclFileNamePortNamesPortTypesPortSerializedTypesPortDirectionsPortWindowSizeEnablesPortWindowMarginEnablesPortBufferSizeEnablesPortBufferMarginEnablesPortSynchronicityEnablesPortSignalSizeEnablesPortBufferSizesPortBufferMarginsFunctionDeclFunctionTemplateSpecKindFunctionTemplateParamNamesFunctionTemplateParamKindsFunctionTemplateParamTypesFunctionTemplateParamValuesFunctionTemplateParamEnablesClassDeclClassTemplateSpecKindClassTemplateParamNamesClassTemplateParamKindsClassTemplateParamTypesClassTemplateParamValuesClassTemplateParamEnablesClassCtorDeclsClassCtorParamNamesClassCtorParamTypesClassCtorParamSerializedTypes[1 1]@C[32 1]@t21@exp_calc_float_lookupt22@../../exp_calc_float.hC[2 1]@t9@cb_input1t10@cb_output1C[2 1]@t38@adf::input_buffer< cfloat > & restrictt31@output_stream_cfloat * restrictC[2 1]@t42@{Q2{R{Tadf::input_buffer{1{t{Scfloat}}}}}}t38@{Q2{P{Toutput_stream{1{t{Scfloat}}}}}}C[2 1]@t5@inputt6@outputC[2 1]@l1@l0@C[2 1]@l1@l0@C[2 1]@l1@l0@C[2 1]@l0@l0@C[2 1]@l1@l0@C[2 1]@l0@l1@C[2 1]@nnC[2 1]@nnt159@template < unsigned int PHASE_INDEX > 
      | void exp_calc_float_lookup(adf::input_buffer< cfloat > & restrict cb_input1, output_stream_cfloat * restrict cb_output1)t8@implicitC[1 1]@t11@PHASE_INDEXC[1 1]@t7@nontypeC[1 1]@t12@unsigned intC[1 1]@nC[1 1]@l1@nne[0 1]@e[0 1]@e[0 1]@e[0 1]@e[0 1]@e[0 1]@e[0 1]@e[0 1]@e[0 1]@
      FunctionDeclTypeOptions=|
      | C[1 1]@t160@template < unsigned int PHASE_INDEX > 
      | void exp_calc_float_lookup(adf::input_buffer< cfloat > && restrict cb_input1, output_stream_cfloat * restrict cb_output1)
      FunctionDecl=|
      | template < unsigned int PHASE_INDEX > 
      | void exp_calc_float_lookup(adf::input_buffer< cfloat > && restrict cb_input1, output_stream_cfloat * restrict cb_output1)
  exp_calc_LUT5 : aieBasic/AIE Kernel  KernelAllAttrs=|  PortNames={'cb_input1'; 'cb_output1'}  PortSerializedTypes={'{Q2{R{Tadf::input_buffer{1{t{Scfloat}}}}}}'; '{Q2{P{Toutput_stream{1{t{Scfloat}}}}}}'}  PortWindowSizes={1.024000000000000000e+03, 0.000000000000000000e+00}  PortWindowMargins={0.000000000000000000e+00, 0.000000000000000000e+00}  PortSynchronicities={'sync', 'auto'}  PortSignalSizes={0.000000000000000000e+00; 1.024000000000000000e+03}  FunctionTemplateSpecKind=implicit  FunctionTemplateParamNames={'PHASE_INDEX'}  FunctionTemplateParamKinds={'nontype'}  FunctionTemplateParamTypes={'unsigned int'}  FunctionTemplateParamValues={'5'}  FunctionIndex=1  FunctionTabVisible=on  FunctionTemplateParamsVisible=on  FunctionDeclTypeOptions=|  FunctionDecl=|  FunctionTemplateParams={ 'PHASE_INDEX', 'unsigned int', '5' }  FunctionTemplateParamsEnables={'off', 'off', 'on'}  PortAttrs={ 'input', 'cb_input1', 'adf::input_buffer< cfloat > & restrict', '1024', '0', 'sync', ''; 'output', 'cb_output1', 'output_stream_cfloat * restrict', '', '', '', '1024' }  PortAttrsEnables={'off', 'off', 'off', 'on', 'off', 'off', 'off';'off', 'off', 'off', 'off', 'off', 'off', 'on'}  SampleTime=-1  KernelHeaderFile=exp_calc_float.h  KernelFunction=exp_calc_float_lookup  KernelSourceFile=exp_calc_float.cc  KernelSearchPaths={}  PreProcOptions={}  blockJsonConstraints=[]
      KernelAllAttrs=|
      | s[12;12;9;9;19;14;21;23;21;23;24;21;15;17;12;24;26;26;26;27;28;9;21;23;23;23;24;25;14;19;19;29]@FunctionNameDeclFileNamePortNamesPortTypesPortSerializedTypesPortDirectionsPortWindowSizeEnablesPortWindowMarginEnablesPortBufferSizeEnablesPortBufferMarginEnablesPortSynchronicityEnablesPortSignalSizeEnablesPortBufferSizesPortBufferMarginsFunctionDeclFunctionTemplateSpecKindFunctionTemplateParamNamesFunctionTemplateParamKindsFunctionTemplateParamTypesFunctionTemplateParamValuesFunctionTemplateParamEnablesClassDeclClassTemplateSpecKindClassTemplateParamNamesClassTemplateParamKindsClassTemplateParamTypesClassTemplateParamValuesClassTemplateParamEnablesClassCtorDeclsClassCtorParamNamesClassCtorParamTypesClassCtorParamSerializedTypes[1 1]@C[32 1]@t21@exp_calc_float_lookupt22@../../exp_calc_float.hC[2 1]@t9@cb_input1t10@cb_output1C[2 1]@t38@adf::input_buffer< cfloat > & restrictt31@output_stream_cfloat * restrictC[2 1]@t42@{Q2{R{Tadf::input_buffer{1{t{Scfloat}}}}}}t38@{Q2{P{Toutput_stream{1{t{Scfloat}}}}}}C[2 1]@t5@inputt6@outputC[2 1]@l1@l0@C[2 1]@l1@l0@C[2 1]@l1@l0@C[2 1]@l0@l0@C[2 1]@l1@l0@C[2 1]@l0@l1@C[2 1]@nnC[2 1]@nnt159@template < unsigned int PHASE_INDEX > 
      | void exp_calc_float_lookup(adf::input_buffer< cfloat > & restrict cb_input1, output_stream_cfloat * restrict cb_output1)t8@implicitC[1 1]@t11@PHASE_INDEXC[1 1]@t7@nontypeC[1 1]@t12@unsigned intC[1 1]@nC[1 1]@l1@nne[0 1]@e[0 1]@e[0 1]@e[0 1]@e[0 1]@e[0 1]@e[0 1]@e[0 1]@e[0 1]@
      FunctionDeclTypeOptions=|
      | C[1 1]@t160@template < unsigned int PHASE_INDEX > 
      | void exp_calc_float_lookup(adf::input_buffer< cfloat > && restrict cb_input1, output_stream_cfloat * restrict cb_output1)
      FunctionDecl=|
      | template < unsigned int PHASE_INDEX > 
      | void exp_calc_float_lookup(adf::input_buffer< cfloat > && restrict cb_input1, output_stream_cfloat * restrict cb_output1)
  exp_calc_LUT6 : aieBasic/AIE Kernel  KernelAllAttrs=|  PortNames={'cb_input1'; 'cb_output1'}  PortSerializedTypes={'{Q2{R{Tadf::input_buffer{1{t{Scfloat}}}}}}'; '{Q2{P{Toutput_stream{1{t{Scfloat}}}}}}'}  PortWindowSizes={1.024000000000000000e+03, 0.000000000000000000e+00}  PortWindowMargins={0.000000000000000000e+00, 0.000000000000000000e+00}  PortSynchronicities={'sync', 'auto'}  PortSignalSizes={0.000000000000000000e+00; 1.024000000000000000e+03}  FunctionTemplateSpecKind=implicit  FunctionTemplateParamNames={'PHASE_INDEX'}  FunctionTemplateParamKinds={'nontype'}  FunctionTemplateParamTypes={'unsigned int'}  FunctionTemplateParamValues={'6'}  FunctionIndex=1  FunctionTabVisible=on  FunctionTemplateParamsVisible=on  FunctionDeclTypeOptions=|  FunctionDecl=|  FunctionTemplateParams={ 'PHASE_INDEX', 'unsigned int', '6' }  FunctionTemplateParamsEnables={'off', 'off', 'on'}  PortAttrs={ 'input', 'cb_input1', 'adf::input_buffer< cfloat > & restrict', '1024', '0', 'sync', ''; 'output', 'cb_output1', 'output_stream_cfloat * restrict', '', '', '', '1024' }  PortAttrsEnables={'off', 'off', 'off', 'on', 'off', 'off', 'off';'off', 'off', 'off', 'off', 'off', 'off', 'on'}  SampleTime=-1  KernelHeaderFile=exp_calc_float.h  KernelFunction=exp_calc_float_lookup  KernelSourceFile=exp_calc_float.cc  KernelSearchPaths={}  PreProcOptions={}  blockJsonConstraints=[]
      KernelAllAttrs=|
      | s[12;12;9;9;19;14;21;23;21;23;24;21;15;17;12;24;26;26;26;27;28;9;21;23;23;23;24;25;14;19;19;29]@FunctionNameDeclFileNamePortNamesPortTypesPortSerializedTypesPortDirectionsPortWindowSizeEnablesPortWindowMarginEnablesPortBufferSizeEnablesPortBufferMarginEnablesPortSynchronicityEnablesPortSignalSizeEnablesPortBufferSizesPortBufferMarginsFunctionDeclFunctionTemplateSpecKindFunctionTemplateParamNamesFunctionTemplateParamKindsFunctionTemplateParamTypesFunctionTemplateParamValuesFunctionTemplateParamEnablesClassDeclClassTemplateSpecKindClassTemplateParamNamesClassTemplateParamKindsClassTemplateParamTypesClassTemplateParamValuesClassTemplateParamEnablesClassCtorDeclsClassCtorParamNamesClassCtorParamTypesClassCtorParamSerializedTypes[1 1]@C[32 1]@t21@exp_calc_float_lookupt22@../../exp_calc_float.hC[2 1]@t9@cb_input1t10@cb_output1C[2 1]@t38@adf::input_buffer< cfloat > & restrictt31@output_stream_cfloat * restrictC[2 1]@t42@{Q2{R{Tadf::input_buffer{1{t{Scfloat}}}}}}t38@{Q2{P{Toutput_stream{1{t{Scfloat}}}}}}C[2 1]@t5@inputt6@outputC[2 1]@l1@l0@C[2 1]@l1@l0@C[2 1]@l1@l0@C[2 1]@l0@l0@C[2 1]@l1@l0@C[2 1]@l0@l1@C[2 1]@nnC[2 1]@nnt159@template < unsigned int PHASE_INDEX > 
      | void exp_calc_float_lookup(adf::input_buffer< cfloat > & restrict cb_input1, output_stream_cfloat * restrict cb_output1)t8@implicitC[1 1]@t11@PHASE_INDEXC[1 1]@t7@nontypeC[1 1]@t12@unsigned intC[1 1]@nC[1 1]@l1@nne[0 1]@e[0 1]@e[0 1]@e[0 1]@e[0 1]@e[0 1]@e[0 1]@e[0 1]@e[0 1]@
      FunctionDeclTypeOptions=|
      | C[1 1]@t160@template < unsigned int PHASE_INDEX > 
      | void exp_calc_float_lookup(adf::input_buffer< cfloat > && restrict cb_input1, output_stream_cfloat * restrict cb_output1)
      FunctionDecl=|
      | template < unsigned int PHASE_INDEX > 
      | void exp_calc_float_lookup(adf::input_buffer< cfloat > && restrict cb_input1, output_stream_cfloat * restrict cb_output1)
  exp_calc_LUT7 : aieBasic/AIE Kernel  KernelAllAttrs=|  PortNames={'cb_input1'; 'cb_output1'}  PortSerializedTypes={'{Q2{R{Tadf::input_buffer{1{t{Scfloat}}}}}}'; '{Q2{P{Toutput_stream{1{t{Scfloat}}}}}}'}  PortWindowSizes={1.024000000000000000e+03, 0.000000000000000000e+00}  PortWindowMargins={0.000000000000000000e+00, 0.000000000000000000e+00}  PortSynchronicities={'sync', 'auto'}  PortSignalSizes={0.000000000000000000e+00; 1.024000000000000000e+03}  FunctionTemplateSpecKind=implicit  FunctionTemplateParamNames={'PHASE_INDEX'}  FunctionTemplateParamKinds={'nontype'}  FunctionTemplateParamTypes={'unsigned int'}  FunctionTemplateParamValues={'7'}  FunctionIndex=1  FunctionTabVisible=on  FunctionTemplateParamsVisible=on  FunctionDeclTypeOptions=|  FunctionDecl=|  FunctionTemplateParams={ 'PHASE_INDEX', 'unsigned int', '7' }  FunctionTemplateParamsEnables={'off', 'off', 'on'}  PortAttrs={ 'input', 'cb_input1', 'adf::input_buffer< cfloat > & restrict', '1024', '0', 'sync', ''; 'output', 'cb_output1', 'output_stream_cfloat * restrict', '', '', '', '1024' }  PortAttrsEnables={'off', 'off', 'off', 'on', 'off', 'off', 'off';'off', 'off', 'off', 'off', 'off', 'off', 'on'}  SampleTime=-1  KernelHeaderFile=exp_calc_float.h  KernelFunction=exp_calc_float_lookup  KernelSourceFile=exp_calc_float.cc  KernelSearchPaths={}  PreProcOptions={}  blockJsonConstraints=[]
      KernelAllAttrs=|
      | s[12;12;9;9;19;14;21;23;21;23;24;21;15;17;12;24;26;26;26;27;28;9;21;23;23;23;24;25;14;19;19;29]@FunctionNameDeclFileNamePortNamesPortTypesPortSerializedTypesPortDirectionsPortWindowSizeEnablesPortWindowMarginEnablesPortBufferSizeEnablesPortBufferMarginEnablesPortSynchronicityEnablesPortSignalSizeEnablesPortBufferSizesPortBufferMarginsFunctionDeclFunctionTemplateSpecKindFunctionTemplateParamNamesFunctionTemplateParamKindsFunctionTemplateParamTypesFunctionTemplateParamValuesFunctionTemplateParamEnablesClassDeclClassTemplateSpecKindClassTemplateParamNamesClassTemplateParamKindsClassTemplateParamTypesClassTemplateParamValuesClassTemplateParamEnablesClassCtorDeclsClassCtorParamNamesClassCtorParamTypesClassCtorParamSerializedTypes[1 1]@C[32 1]@t21@exp_calc_float_lookupt22@../../exp_calc_float.hC[2 1]@t9@cb_input1t10@cb_output1C[2 1]@t38@adf::input_buffer< cfloat > & restrictt31@output_stream_cfloat * restrictC[2 1]@t42@{Q2{R{Tadf::input_buffer{1{t{Scfloat}}}}}}t38@{Q2{P{Toutput_stream{1{t{Scfloat}}}}}}C[2 1]@t5@inputt6@outputC[2 1]@l1@l0@C[2 1]@l1@l0@C[2 1]@l1@l0@C[2 1]@l0@l0@C[2 1]@l1@l0@C[2 1]@l0@l1@C[2 1]@nnC[2 1]@nnt159@template < unsigned int PHASE_INDEX > 
      | void exp_calc_float_lookup(adf::input_buffer< cfloat > & restrict cb_input1, output_stream_cfloat * restrict cb_output1)t8@implicitC[1 1]@t11@PHASE_INDEXC[1 1]@t7@nontypeC[1 1]@t12@unsigned intC[1 1]@nC[1 1]@l1@nne[0 1]@e[0 1]@e[0 1]@e[0 1]@e[0 1]@e[0 1]@e[0 1]@e[0 1]@e[0 1]@
      FunctionDeclTypeOptions=|
      | C[1 1]@t160@template < unsigned int PHASE_INDEX > 
      | void exp_calc_float_lookup(adf::input_buffer< cfloat > && restrict cb_input1, output_stream_cfloat * restrict cb_output1)
      FunctionDecl=|
      | template < unsigned int PHASE_INDEX > 
      | void exp_calc_float_lookup(adf::input_buffer< cfloat > && restrict cb_input1, output_stream_cfloat * restrict cb_output1)
  exp_calc_LUT8 : aieBasic/AIE Kernel  KernelAllAttrs=|  PortNames={'cb_input1'; 'cb_output1'}  PortSerializedTypes={'{Q2{R{Tadf::input_buffer{1{t{Scfloat}}}}}}'; '{Q2{P{Toutput_stream{1{t{Scfloat}}}}}}'}  PortWindowSizes={1.024000000000000000e+03, 0.000000000000000000e+00}  PortWindowMargins={0.000000000000000000e+00, 0.000000000000000000e+00}  PortSynchronicities={'sync', 'auto'}  PortSignalSizes={0.000000000000000000e+00; 1.024000000000000000e+03}  FunctionTemplateSpecKind=implicit  FunctionTemplateParamNames={'PHASE_INDEX'}  FunctionTemplateParamKinds={'nontype'}  FunctionTemplateParamTypes={'unsigned int'}  FunctionTemplateParamValues={'8'}  FunctionIndex=1  FunctionTabVisible=on  FunctionTemplateParamsVisible=on  FunctionDeclTypeOptions=|  FunctionDecl=|  FunctionTemplateParams={ 'PHASE_INDEX', 'unsigned int', '8' }  FunctionTemplateParamsEnables={'off', 'off', 'on'}  PortAttrs={ 'input', 'cb_input1', 'adf::input_buffer< cfloat > & restrict', '1024', '0', 'sync', ''; 'output', 'cb_output1', 'output_stream_cfloat * restrict', '', '', '', '1024' }  PortAttrsEnables={'off', 'off', 'off', 'on', 'off', 'off', 'off';'off', 'off', 'off', 'off', 'off', 'off', 'on'}  SampleTime=-1  KernelHeaderFile=exp_calc_float.h  KernelFunction=exp_calc_float_lookup  KernelSourceFile=exp_calc_float.cc  KernelSearchPaths={}  PreProcOptions={}  blockJsonConstraints=[]
      KernelAllAttrs=|
      | s[12;12;9;9;19;14;21;23;21;23;24;21;15;17;12;24;26;26;26;27;28;9;21;23;23;23;24;25;14;19;19;29]@FunctionNameDeclFileNamePortNamesPortTypesPortSerializedTypesPortDirectionsPortWindowSizeEnablesPortWindowMarginEnablesPortBufferSizeEnablesPortBufferMarginEnablesPortSynchronicityEnablesPortSignalSizeEnablesPortBufferSizesPortBufferMarginsFunctionDeclFunctionTemplateSpecKindFunctionTemplateParamNamesFunctionTemplateParamKindsFunctionTemplateParamTypesFunctionTemplateParamValuesFunctionTemplateParamEnablesClassDeclClassTemplateSpecKindClassTemplateParamNamesClassTemplateParamKindsClassTemplateParamTypesClassTemplateParamValuesClassTemplateParamEnablesClassCtorDeclsClassCtorParamNamesClassCtorParamTypesClassCtorParamSerializedTypes[1 1]@C[32 1]@t21@exp_calc_float_lookupt22@../../exp_calc_float.hC[2 1]@t9@cb_input1t10@cb_output1C[2 1]@t38@adf::input_buffer< cfloat > & restrictt31@output_stream_cfloat * restrictC[2 1]@t42@{Q2{R{Tadf::input_buffer{1{t{Scfloat}}}}}}t38@{Q2{P{Toutput_stream{1{t{Scfloat}}}}}}C[2 1]@t5@inputt6@outputC[2 1]@l1@l0@C[2 1]@l1@l0@C[2 1]@l1@l0@C[2 1]@l0@l0@C[2 1]@l1@l0@C[2 1]@l0@l1@C[2 1]@nnC[2 1]@nnt159@template < unsigned int PHASE_INDEX > 
      | void exp_calc_float_lookup(adf::input_buffer< cfloat > & restrict cb_input1, output_stream_cfloat * restrict cb_output1)t8@implicitC[1 1]@t11@PHASE_INDEXC[1 1]@t7@nontypeC[1 1]@t12@unsigned intC[1 1]@nC[1 1]@l1@nne[0 1]@e[0 1]@e[0 1]@e[0 1]@e[0 1]@e[0 1]@e[0 1]@e[0 1]@e[0 1]@
      FunctionDeclTypeOptions=|
      | C[1 1]@t160@template < unsigned int PHASE_INDEX > 
      | void exp_calc_float_lookup(adf::input_buffer< cfloat > && restrict cb_input1, output_stream_cfloat * restrict cb_output1)
      FunctionDecl=|
      | template < unsigned int PHASE_INDEX > 
      | void exp_calc_float_lookup(adf::input_buffer< cfloat > && restrict cb_input1, output_stream_cfloat * restrict cb_output1)
  exp_calc_LUT9 : aieBasic/AIE Kernel  KernelAllAttrs=|  PortNames={'cb_input1'; 'cb_output1'}  PortSerializedTypes={'{Q2{R{Tadf::input_buffer{1{t{Scfloat}}}}}}'; '{Q2{P{Toutput_stream{1{t{Scfloat}}}}}}'}  PortWindowSizes={1.024000000000000000e+03, 0.000000000000000000e+00}  PortWindowMargins={0.000000000000000000e+00, 0.000000000000000000e+00}  PortSynchronicities={'sync', 'auto'}  PortSignalSizes={0.000000000000000000e+00; 1.024000000000000000e+03}  FunctionTemplateSpecKind=implicit  FunctionTemplateParamNames={'PHASE_INDEX'}  FunctionTemplateParamKinds={'nontype'}  FunctionTemplateParamTypes={'unsigned int'}  FunctionTemplateParamValues={'9'}  FunctionIndex=1  FunctionTabVisible=on  FunctionTemplateParamsVisible=on  FunctionDeclTypeOptions=|  FunctionDecl=|  FunctionTemplateParams={ 'PHASE_INDEX', 'unsigned int', '9' }  FunctionTemplateParamsEnables={'off', 'off', 'on'}  PortAttrs={ 'input', 'cb_input1', 'adf::input_buffer< cfloat > & restrict', '1024', '0', 'sync', ''; 'output', 'cb_output1', 'output_stream_cfloat * restrict', '', '', '', '1024' }  PortAttrsEnables={'off', 'off', 'off', 'on', 'off', 'off', 'off';'off', 'off', 'off', 'off', 'off', 'off', 'on'}  SampleTime=-1  KernelHeaderFile=exp_calc_float.h  KernelFunction=exp_calc_float_lookup  KernelSourceFile=exp_calc_float.cc  KernelSearchPaths={}  PreProcOptions={}  blockJsonConstraints=[]
      KernelAllAttrs=|
      | s[12;12;9;9;19;14;21;23;21;23;24;21;15;17;12;24;26;26;26;27;28;9;21;23;23;23;24;25;14;19;19;29]@FunctionNameDeclFileNamePortNamesPortTypesPortSerializedTypesPortDirectionsPortWindowSizeEnablesPortWindowMarginEnablesPortBufferSizeEnablesPortBufferMarginEnablesPortSynchronicityEnablesPortSignalSizeEnablesPortBufferSizesPortBufferMarginsFunctionDeclFunctionTemplateSpecKindFunctionTemplateParamNamesFunctionTemplateParamKindsFunctionTemplateParamTypesFunctionTemplateParamValuesFunctionTemplateParamEnablesClassDeclClassTemplateSpecKindClassTemplateParamNamesClassTemplateParamKindsClassTemplateParamTypesClassTemplateParamValuesClassTemplateParamEnablesClassCtorDeclsClassCtorParamNamesClassCtorParamTypesClassCtorParamSerializedTypes[1 1]@C[32 1]@t21@exp_calc_float_lookupt22@../../exp_calc_float.hC[2 1]@t9@cb_input1t10@cb_output1C[2 1]@t38@adf::input_buffer< cfloat > & restrictt31@output_stream_cfloat * restrictC[2 1]@t42@{Q2{R{Tadf::input_buffer{1{t{Scfloat}}}}}}t38@{Q2{P{Toutput_stream{1{t{Scfloat}}}}}}C[2 1]@t5@inputt6@outputC[2 1]@l1@l0@C[2 1]@l1@l0@C[2 1]@l1@l0@C[2 1]@l0@l0@C[2 1]@l1@l0@C[2 1]@l0@l1@C[2 1]@nnC[2 1]@nnt159@template < unsigned int PHASE_INDEX > 
      | void exp_calc_float_lookup(adf::input_buffer< cfloat > & restrict cb_input1, output_stream_cfloat * restrict cb_output1)t8@implicitC[1 1]@t11@PHASE_INDEXC[1 1]@t7@nontypeC[1 1]@t12@unsigned intC[1 1]@nC[1 1]@l1@nne[0 1]@e[0 1]@e[0 1]@e[0 1]@e[0 1]@e[0 1]@e[0 1]@e[0 1]@e[0 1]@
      FunctionDeclTypeOptions=|
      | C[1 1]@t160@template < unsigned int PHASE_INDEX > 
      | void exp_calc_float_lookup(adf::input_buffer< cfloat > && restrict cb_input1, output_stream_cfloat * restrict cb_output1)
      FunctionDecl=|
      | template < unsigned int PHASE_INDEX > 
      | void exp_calc_float_lookup(adf::input_buffer< cfloat > && restrict cb_input1, output_stream_cfloat * restrict cb_output1)
  Out1 : Outport
  Out2 : Outport  Port=2
  Out3 : Outport  Port=3
  Out4 : Outport  Port=4
  Out5 : Outport  Port=5
  Out6 : Outport  Port=6
  Out7 : Outport  Port=7
  Out8 : Outport  Port=8
  Out9 : Outport  Port=9
  Out10 : Outport  Port=10
  Out11 : Outport  Port=11
  Out12 : Outport  Port=12
  Out13 : Outport  Port=13
  Out14 : Outport  Port=14
  Out15 : Outport  Port=15
  Out16 : Outport  Port=16
  Out17 : Outport  Port=17
  Out18 : Outport  Port=18
  Out19 : Outport  Port=19
  Out20 : Outport  Port=20
  Out21 : Outport  Port=21
  Out22 : Outport  Port=22
  Out23 : Outport  Port=23
  Out24 : Outport  Port=24
  Out25 : Outport  Port=25
  Out26 : Outport  Port=26
  Out27 : Outport  Port=27
  Out28 : Outport  Port=28
  Out29 : Outport  Port=29
  Out30 : Outport  Port=30
  Out31 : Outport  Port=31
  Out32 : Outport  Port=32
  wires:
  In5/1 -> PLIO4/1
  In13/1 -> PLIO12/1
  In6/1 -> PLIO5/1
  In11/1 -> PLIO10/1
  In12/1 -> PLIO11/1
  In16/1 -> PLIO15/1
  In14/1 -> PLIO13/1
  In8/1 -> PLIO7/1
  In3/1 -> PLIO2/1
  In4/1 -> PLIO3/1
  In10/1 -> PLIO9/1
  In7/1 -> PLIO6/1
  In9/1 -> PLIO8/1
  In2/1 -> PLIO1/1
  In15/1 -> PLIO14/1
  In1/1 -> PLIO/1
  PLIO/1 -> FFT/1
  FFT/1 -> PLIO32/1
  In17/1 -> PLIO16/1
  In31/1 -> PLIO22/1
  In18/1 -> PLIO17/1
  In25/1 -> PLIO30/1
  In23/1 -> PLIO28/1
  In26/1 -> PLIO31/1
  In20/1 -> PLIO25/1
  In19/1 -> PLIO24/1
  In24/1 -> PLIO29/1
  In30/1 -> PLIO21/1
  In32/1 -> PLIO23/1
  In28/1 -> PLIO19/1
  In27/1 -> PLIO18/1
  In22/1 -> PLIO27/1
  In29/1 -> PLIO20/1
  In21/1 -> PLIO26/1
  PLIO58/1 -> Out5/1
  PLIO55/1 -> Out4/1
  PLIO38/1 -> Out15/1
  PLIO36/1 -> Out13/1
  PLIO60/1 -> Out7/1
  PLIO33/1 -> Out2/1
  PLIO61/1 -> Out8/1
  PLIO34/1 -> Out11/1
  PLIO37/1 -> Out14/1
  PLIO59/1 -> Out6/1
  PLIO44/1 -> Out3/1
  PLIO39/1 -> Out16/1
  PLIO62/1 -> Out9/1
  PLIO35/1 -> Out12/1
  PLIO63/1 -> Out10/1
  PLIO32/1 -> Out1/1
  PLIO40/1 -> Out17/1
  PLIO41/1 -> Out18/1
  PLIO49/1 -> Out19/1
  PLIO50/1 -> Out20/1
  PLIO51/1 -> Out21/1
  PLIO52/1 -> Out22/1
  PLIO53/1 -> Out23/1
  PLIO54/1 -> Out24/1
  PLIO56/1 -> Out25/1
  PLIO57/1 -> Out26/1
  PLIO42/1 -> Out27/1
  PLIO43/1 -> Out28/1
  PLIO45/1 -> Out29/1
  PLIO46/1 -> Out30/1
  PLIO47/1 -> Out31/1
  PLIO48/1 -> Out32/1
  PLIO21/1 -> FFT21/1
  PLIO22/1 -> FFT22/1
  PLIO17/1 -> FFT17/1
  PLIO19/1 -> FFT19/1
  PLIO14/1 -> FFT14/1
  PLIO11/1 -> FFT11/1
  PLIO8/1 -> FFT8/1
  PLIO1/1 -> FFT1/1
  PLIO3/1 -> FFT3/1
  PLIO13/1 -> FFT13/1
  PLIO2/1 -> FFT2/1
  PLIO30/1 -> FFT30/1
  PLIO18/1 -> FFT18/1
  PLIO5/1 -> FFT5/1
  PLIO27/1 -> FFT27/1
  PLIO7/1 -> FFT7/1
  PLIO6/1 -> FFT6/1
  PLIO25/1 -> FFT25/1
  PLIO26/1 -> FFT26/1
  PLIO31/1 -> FFT31/1
  PLIO15/1 -> FFT15/1
  PLIO29/1 -> FFT29/1
  PLIO4/1 -> FFT4/1
  PLIO9/1 -> FFT9/1
  PLIO23/1 -> FFT23/1
  PLIO16/1 -> FFT16/1
  PLIO20/1 -> FFT20/1
  PLIO12/1 -> FFT12/1
  PLIO24/1 -> FFT24/1
  PLIO28/1 -> FFT28/1
  PLIO10/1 -> FFT10/1
  FFT23/1 -> exp_calc_LUT31/1
  FFT22/1 -> exp_calc_LUT30/1
  FFT21/1 -> exp_calc_LUT29/1
  FFT20/1 -> exp_calc_LUT28/1
  FFT19/1 -> exp_calc_LUT27/1
  FFT18/1 -> exp_calc_LUT26/1
  FFT31/1 -> exp_calc_LUT25/1
  FFT30/1 -> exp_calc_LUT24/1
  FFT29/1 -> exp_calc_LUT23/1
  FFT28/1 -> exp_calc_LUT22/1
  FFT27/1 -> exp_calc_LUT21/1
  FFT26/1 -> exp_calc_LUT20/1
  FFT25/1 -> exp_calc_LUT19/1
  FFT24/1 -> exp_calc_LUT18/1
  FFT17/1 -> exp_calc_LUT17/1
  FFT16/1 -> exp_calc_LUT16/1
  FFT8/1 -> exp_calc_LUT8/1
  FFT7/1 -> exp_calc_LUT7/1
  FFT6/1 -> exp_calc_LUT6/1
  FFT5/1 -> exp_calc_LUT5/1
  FFT4/1 -> exp_calc_LUT4/1
  FFT3/1 -> exp_calc_LUT3/1
  FFT2/1 -> exp_calc_LUT2/1
  FFT1/1 -> exp_calc_LUT1/1
  FFT9/1 -> exp_calc_LUT9/1
  FFT10/1 -> exp_calc_LUT10/1
  FFT11/1 -> exp_calc_LUT11/1
  FFT12/1 -> exp_calc_LUT12/1
  FFT13/1 -> exp_calc_LUT13/1
  FFT14/1 -> exp_calc_LUT14/1
  FFT15/1 -> exp_calc_LUT15/1
  exp_calc_LUT15/1 -> PLIO39/1
  exp_calc_LUT18/1 -> PLIO49/1
  exp_calc_LUT26/1 -> PLIO42/1
  exp_calc_LUT8/1 -> PLIO62/1
  exp_calc_LUT22/1 -> PLIO53/1
  exp_calc_LUT7/1 -> PLIO61/1
  exp_calc_LUT5/1 -> PLIO59/1
  exp_calc_LUT19/1 -> PLIO50/1
  exp_calc_LUT23/1 -> PLIO54/1
  exp_calc_LUT6/1 -> PLIO60/1
  exp_calc_LUT11/1 -> PLIO35/1
  exp_calc_LUT9/1 -> PLIO63/1
  exp_calc_LUT24/1 -> PLIO56/1
  exp_calc_LUT10/1 -> PLIO34/1
  exp_calc_LUT28/1 -> PLIO45/1
  exp_calc_LUT31/1 -> PLIO48/1
  exp_calc_LUT25/1 -> PLIO57/1
  exp_calc_LUT4/1 -> PLIO58/1
  exp_calc_LUT27/1 -> PLIO43/1
  exp_calc_LUT17/1 -> PLIO41/1
  exp_calc_LUT3/1 -> PLIO55/1
  exp_calc_LUT13/1 -> PLIO37/1
  exp_calc_LUT1/1 -> PLIO33/1
  exp_calc_LUT14/1 -> PLIO38/1
  exp_calc_LUT16/1 -> PLIO40/1
  exp_calc_LUT20/1 -> PLIO51/1
  exp_calc_LUT2/1 -> PLIO44/1
  exp_calc_LUT12/1 -> PLIO36/1
  exp_calc_LUT21/1 -> PLIO52/1
  exp_calc_LUT29/1 -> PLIO46/1
  exp_calc_LUT30/1 -> PLIO47/1
